simulink library "outp"  (R2021b)
(part 8 of 10)

  VTPM_LRSensorMode_flg_Inproc : FVT_lib/outp/OverrideAndLimit  SystemSampleTime=-1  VariantActivationTime=update diagram  Latency=0  AutoFrameSizeCalculation=off
      link override Signal_Limit/_maxval: Value=KOUTP_LRSensorMode_flg_maxval
      link override Signal_Limit/_minval: Value=KOUTP_LRSensorMode_flg_minval
      link override Signal_Override/_ovrdflg: Value=KOUTP_LRSensorMode_flg_ovrdflg
      link override Signal_Override/_ovrdval: Value=KOUTP_LRSensorMode_flg_ovrdval
  VTPM_LRWheelDebug_flg_Inproc : FVT_lib/outp/OverrideAndLimit  SystemSampleTime=-1  VariantActivationTime=update diagram  Latency=0  AutoFrameSizeCalculation=off
      link override Signal_Limit/_maxval: Value=KOUTP_LRWheelDebug_flg_maxval
      link override Signal_Limit/_minval: Value=KOUTP_LRWheelDebug_flg_minval
      link override Signal_Override/_ovrdflg: Value=KOUTP_LRWheelDebug_flg_ovrdflg
      link override Signal_Override/_ovrdval: Value=KOUTP_LRWheelDebug_flg_ovrdval
  VTPM_LRWheelPSW_raw8_Inproc : FVT_lib/outp/OverrideAndLimit  SystemSampleTime=-1  VariantActivationTime=update diagram  Latency=0  AutoFrameSizeCalculation=off
      link override Signal_Limit/_maxval: Value=KOUTP_LRWheelPSW_raw8_maxval
      link override Signal_Limit/_minval: Value=KOUTP_LRWheelPSW_raw8_minval
      link override Signal_Override/_ovrdflg: Value=KOUTP_LRWheelPSW_raw8_ovrdflg
      link override Signal_Override/_ovrdval: Value=KOUTP_LRWheelPSW_raw8_ovrdval
  VTPM_LRWheelPress_raw8_Inproc : FVT_lib/outp/OverrideAndLimit  SystemSampleTime=-1  VariantActivationTime=update diagram  Latency=0  AutoFrameSizeCalculation=off
      link override Signal_Limit/_maxval: Value=KOUTP_LRWheelPress_raw8_maxval
      link override Signal_Limit/_minval: Value=KOUTP_LRWheelPress_raw8_minval
      link override Signal_Override/_ovrdflg: Value=KOUTP_LRWheelPress_raw8_ovrdflg
      link override Signal_Override/_ovrdval: Value=KOUTP_LRWheelPress_raw8_ovrdval
  VTPM_LRWheelTemp_C_Inproc : FVT_lib/outp/OverrideAndLimit  SystemSampleTime=-1  VariantActivationTime=update diagram  Latency=0  AutoFrameSizeCalculation=off
      link override Signal_Limit/_maxval: Value=KOUTP_LRWheelTemp_C_maxval
      link override Signal_Limit/_minval: Value=KOUTP_LRWheelTemp_C_minval
      link override Signal_Override/_ovrdflg: Value=KOUTP_LRWheelTemp_C_ovrdflg
      link override Signal_Override/_ovrdval: Value=KOUTP_LRWheelTemp_C_ovrdval
  VTPM_LRWheelTmpIndi_flg_Inproc : FVT_lib/outp/OverrideAndLimit  SystemSampleTime=-1  VariantActivationTime=update diagram  Latency=0  AutoFrameSizeCalculation=off
      link override Signal_Limit/_maxval: Value=KOUTP_LRWheelTmpIndi_flg_maxval
      link override Signal_Limit/_minval: Value=KOUTP_LRWheelTmpIndi_flg_minval
      link override Signal_Override/_ovrdflg: Value=KOUTP_LRWheelTmpIndi_flg_ovrdflg
      link override Signal_Override/_ovrdval: Value=KOUTP_LRWheelTmpIndi_flg_ovrdval
  VTPM_ModelVersionChksum_raw_Inproc : FVT_lib/outp/OverrideAndLimit  SystemSampleTime=-1  VariantActivationTime=update diagram  Latency=0  AutoFrameSizeCalculation=off
      link override Signal_Limit/_maxval: Value=KOUTP_ModelVersionChksum_raw_maxval
      link override Signal_Limit/_minval: Value=KOUTP_ModelVersionChksum_raw_minval
      link override Signal_Override/_ovrdflg: Value=KOUTP_ModelVersionChksum_raw_ovrdflg
      link override Signal_Override/_ovrdval: Value=KOUTP_ModelVersionChksum_raw_ovrdval
  VTPM_ModelVersion_raw_Inproc : FVT_lib/outp/OverrideAndLimit  SystemSampleTime=-1  VariantActivationTime=update diagram  Latency=0  AutoFrameSizeCalculation=off
      link override Signal_Limit/_maxval: Value=KOUTP_ModelVersion_raw_maxval
      link override Signal_Limit/_minval: Value=KOUTP_ModelVersion_raw_minval
      link override Signal_Override/_ovrdflg: Value=KOUTP_ModelVersion_raw_ovrdflg
      link override Signal_Override/_ovrdval: Value=KOUTP_ModelVersion_raw_ovrdval
  VTPM_Prepresstempvalid_enum_Inproc : FVT_lib/outp/OverrideAndLimit  SystemSampleTime=-1  VariantActivationTime=update diagram  Latency=0  AutoFrameSizeCalculation=off
      link override Signal_Limit/_maxval: Value=KOUTP_Prepresstempvalid_enum_maxval
      link override Signal_Limit/_minval: Value=KOUTP_Prepresstempvalid_enum_minval
      link override Signal_Override/_ovrdflg: Value=KOUTP_Prepresstempvalid_enum_ovrdflg
      link override Signal_Override/_ovrdval: Value=KOUTP_Prepresstempvalid_enum_ovrdval
  VTPM_RFBatWarn_flg_Inproc : FVT_lib/outp/OverrideAndLimit  SystemSampleTime=-1  VariantActivationTime=update diagram  Latency=0  AutoFrameSizeCalculation=off
      link override Signal_Limit/_maxval: Value=KOUTP_RFBatWarn_flg_maxval
      link override Signal_Limit/_minval: Value=KOUTP_RFBatWarn_flg_minval
      link override Signal_Override/_ovrdflg: Value=KOUTP_RFBatWarn_flg_ovrdflg
      link override Signal_Override/_ovrdval: Value=KOUTP_RFBatWarn_flg_ovrdval
  VTPM_RFP20_raw8_Inproc : FVT_lib/outp/OverrideAndLimit  SystemSampleTime=-1  VariantActivationTime=update diagram  Latency=0  AutoFrameSizeCalculation=off
      link override Signal_Limit/_maxval: Value=KOUTP_RFP20_raw8_maxval
      link override Signal_Limit/_minval: Value=KOUTP_RFP20_raw8_minval
      link override Signal_Override/_ovrdflg: Value=KOUTP_RFP20_raw8_ovrdflg
      link override Signal_Override/_ovrdval: Value=KOUTP_RFP20_raw8_ovrdval
  VTPM_RFPind_enum_Inproc : FVT_lib/outp/OverrideAndLimit  SystemSampleTime=-1  VariantActivationTime=update diagram  Latency=0  AutoFrameSizeCalculation=off
      link override Signal_Limit/_maxval: Value=KOUTP_RFPind_enum_maxval
      link override Signal_Limit/_minval: Value=KOUTP_RFPind_enum_minval
      link override Signal_Override/_ovrdflg: Value=KOUTP_RFPind_enum_ovrdflg
      link override Signal_Override/_ovrdval: Value=KOUTP_RFPind_enum_ovrdval
  VTPM_RFPressIndi_enum_Inproc : FVT_lib/outp/OverrideAndLimit  SystemSampleTime=-1  VariantActivationTime=update diagram  Latency=0  AutoFrameSizeCalculation=off
      link override Signal_Limit/_maxval: Value=KOUTP_RFPressIndi_enum_maxval
      link override Signal_Limit/_minval: Value=KOUTP_RFPressIndi_enum_minval
      link override Signal_Override/_ovrdflg: Value=KOUTP_RFPressIndi_enum_ovrdflg
      link override Signal_Override/_ovrdval: Value=KOUTP_RFPressIndi_enum_ovrdval
  VTPM_RFSensorFail_flg_Inproc : FVT_lib/outp/OverrideAndLimit  SystemSampleTime=-1  VariantActivationTime=update diagram  Latency=0  AutoFrameSizeCalculation=off
      link override Signal_Limit/_maxval: Value=KOUTP_RFSensorFail_flg_maxval
      link override Signal_Limit/_minval: Value=KOUTP_RFSensorFail_flg_minval
      link override Signal_Override/_ovrdflg: Value=KOUTP_RFSensorFail_flg_ovrdflg
      link override Signal_Override/_ovrdval: Value=KOUTP_RFSensorFail_flg_ovrdval
  VTPM_RFSensorMode_flg_Inproc : FVT_lib/outp/OverrideAndLimit  SystemSampleTime=-1  VariantActivationTime=update diagram  Latency=0  AutoFrameSizeCalculation=off
      link override Signal_Limit/_maxval: Value=KOUTP_RFSensorMode_flg_maxval
      link override Signal_Limit/_minval: Value=KOUTP_RFSensorMode_flg_minval
      link override Signal_Override/_ovrdflg: Value=KOUTP_RFSensorMode_flg_ovrdflg
      link override Signal_Override/_ovrdval: Value=KOUTP_RFSensorMode_flg_ovrdval
  VTPM_RFWheelDebug_flg_Inproc : FVT_lib/outp/OverrideAndLimit  SystemSampleTime=-1  VariantActivationTime=update diagram  Latency=0  AutoFrameSizeCalculation=off
      link override Signal_Limit/_maxval: Value=KOUTP_RFWheelDebug_flg_maxval
      link override Signal_Limit/_minval: Value=KOUTP_RFWheelDebug_flg_minval
      link override Signal_Override/_ovrdflg: Value=KOUTP_RFWheelDebug_flg_ovrdflg
      link override Signal_Override/_ovrdval: Value=KOUTP_RFWheelDebug_flg_ovrdval
  VTPM_RFWheelPSW_raw8_Inproc : FVT_lib/outp/OverrideAndLimit  SystemSampleTime=-1  VariantActivationTime=update diagram  Latency=0  AutoFrameSizeCalculation=off
      link override Signal_Limit/_maxval: Value=KOUTP_RFWheelPSW_raw8_maxval
      link override Signal_Limit/_minval: Value=KOUTP_RFWheelPSW_raw8_minval
      link override Signal_Override/_ovrdflg: Value=KOUTP_RFWheelPSW_raw8_ovrdflg
      link override Signal_Override/_ovrdval: Value=KOUTP_RFWheelPSW_raw8_ovrdval
  VTPM_RFWheelPress_raw8_Inproc : FVT_lib/outp/OverrideAndLimit  SystemSampleTime=-1  VariantActivationTime=update diagram  Latency=0  AutoFrameSizeCalculation=off
      link override Signal_Limit/_maxval: Value=KOUTP_RFWheelPress_raw8_maxval
      link override Signal_Limit/_minval: Value=KOUTP_RFWheelPress_raw8_minval
      link override Signal_Override/_ovrdflg: Value=KOUTP_RFWheelPress_raw8_ovrdflg
      link override Signal_Override/_ovrdval: Value=KOUTP_RFWheelPress_raw8_ovrdval
  VTPM_RFWheelTemp_C_Inproc : FVT_lib/outp/OverrideAndLimit  SystemSampleTime=-1  VariantActivationTime=update diagram  Latency=0  AutoFrameSizeCalculation=off
      link override Signal_Limit/_maxval: Value=KOUTP_RFWheelTemp_C_maxval
      link override Signal_Limit/_minval: Value=KOUTP_RFWheelTemp_C_minval
      link override Signal_Override/_ovrdflg: Value=KOUTP_RFWheelTemp_C_ovrdflg
      link override Signal_Override/_ovrdval: Value=KOUTP_RFWheelTemp_C_ovrdval
  VTPM_RFWheelTmpIndi_flg_Inproc : FVT_lib/outp/OverrideAndLimit  SystemSampleTime=-1  VariantActivationTime=update diagram  Latency=0  AutoFrameSizeCalculation=off
      link override Signal_Limit/_maxval: Value=KOUTP_RFWheelTmpIndi_flg_maxval
      link override Signal_Limit/_minval: Value=KOUTP_RFWheelTmpIndi_flg_minval
      link override Signal_Override/_ovrdflg: Value=KOUTP_RFWheelTmpIndi_flg_ovrdflg
      link override Signal_Override/_ovrdval: Value=KOUTP_RFWheelTmpIndi_flg_ovrdval
  VTPM_RRBatWarn_flg_Inproc : FVT_lib/outp/OverrideAndLimit  SystemSampleTime=-1  VariantActivationTime=update diagram  Latency=0  AutoFrameSizeCalculation=off
      link override Signal_Limit/_maxval: Value=KOUTP_RRBatWarn_flg_maxval
      link override Signal_Limit/_minval: Value=KOUTP_RRBatWarn_flg_minval
      link override Signal_Override/_ovrdflg: Value=KOUTP_RRBatWarn_flg_ovrdflg
      link override Signal_Override/_ovrdval: Value=KOUTP_RRBatWarn_flg_ovrdval
  VTPM_RRP20_raw8_Inproc : FVT_lib/outp/OverrideAndLimit  SystemSampleTime=-1  VariantActivationTime=update diagram  Latency=0  AutoFrameSizeCalculation=off
      link override Signal_Limit/_maxval: Value=KOUTP_RRP20_raw8_maxval
      link override Signal_Limit/_minval: Value=KOUTP_RRP20_raw8_minval
      link override Signal_Override/_ovrdflg: Value=KOUTP_RRP20_raw8_ovrdflg
      link override Signal_Override/_ovrdval: Value=KOUTP_RRP20_raw8_ovrdval
  VTPM_RRPindi_enum_Inproc : FVT_lib/outp/OverrideAndLimit  SystemSampleTime=-1  VariantActivationTime=update diagram  Latency=0  AutoFrameSizeCalculation=off
      link override Signal_Limit/_maxval: Value=KOUTP_RRPindi_enum_maxval
      link override Signal_Limit/_minval: Value=KOUTP_RRPindi_enum_minval
      link override Signal_Override/_ovrdflg: Value=KOUTP_RRPindi_enum_ovrdflg
      link override Signal_Override/_ovrdval: Value=KOUTP_RRPindi_enum_ovrdval
  VTPM_RRPressIndi_enum_Inproc : FVT_lib/outp/OverrideAndLimit  SystemSampleTime=-1  VariantActivationTime=update diagram  Latency=0  AutoFrameSizeCalculation=off
      link override Signal_Limit/_maxval: Value=KOUTP_RRPressIndi_enum_maxval
      link override Signal_Limit/_minval: Value=KOUTP_RRPressIndi_enum_minval
      link override Signal_Override/_ovrdflg: Value=KOUTP_RRPressIndi_enum_ovrdflg
      link override Signal_Override/_ovrdval: Value=KOUTP_RRPressIndi_enum_ovrdval
  VTPM_RRSensorFail_flg_Inproc : FVT_lib/outp/OverrideAndLimit  SystemSampleTime=-1  VariantActivationTime=update diagram  Latency=0  AutoFrameSizeCalculation=off
      link override Signal_Limit/_maxval: Value=KOUTP_RRSensorFail_flg_maxval
      link override Signal_Limit/_minval: Value=KOUTP_RRSensorFail_flg_minval
      link override Signal_Override/_ovrdflg: Value=KOUTP_RRSensorFail_flg_ovrdflg
      link override Signal_Override/_ovrdval: Value=KOUTP_RRSensorFail_flg_ovrdval
  VTPM_RRSensorMode_flg_Inproc : FVT_lib/outp/OverrideAndLimit  SystemSampleTime=-1  VariantActivationTime=update diagram  Latency=0  AutoFrameSizeCalculation=off
      link override Signal_Limit/_maxval: Value=KOUTP_RRSensorMode_flg_maxval
      link override Signal_Limit/_minval: Value=KOUTP_RRSensorMode_flg_minval
      link override Signal_Override/_ovrdflg: Value=KOUTP_RRSensorMode_flg_ovrdflg
      link override Signal_Override/_ovrdval: Value=KOUTP_RRSensorMode_flg_ovrdval
  VTPM_RRWheelDebug_flg_Inproc : FVT_lib/outp/OverrideAndLimit  SystemSampleTime=-1  VariantActivationTime=update diagram  Latency=0  AutoFrameSizeCalculation=off
      link override Signal_Limit/_maxval: Value=KOUTP_RRWheelDebug_flg_maxval
      link override Signal_Limit/_minval: Value=KOUTP_RRWheelDebug_flg_minval
      link override Signal_Override/_ovrdflg: Value=KOUTP_RRWheelDebug_flg_ovrdflg
      link override Signal_Override/_ovrdval: Value=KOUTP_RRWheelDebug_flg_ovrdval
  VTPM_RRWheelPSW_raw8_Inproc : FVT_lib/outp/OverrideAndLimit  SystemSampleTime=-1  VariantActivationTime=update diagram  Latency=0  AutoFrameSizeCalculation=off
      link override Signal_Limit/_maxval: Value=KOUTP_RRWheelPSW_raw8_maxval
      link override Signal_Limit/_minval: Value=KOUTP_RRWheelPSW_raw8_minval
      link override Signal_Override/_ovrdflg: Value=KOUTP_RRWheelPSW_raw8_ovrdflg
      link override Signal_Override/_ovrdval: Value=KOUTP_RRWheelPSW_raw8_ovrdval
  VTPM_RRWheelPress_raw8_Inproc : FVT_lib/outp/OverrideAndLimit  SystemSampleTime=-1  VariantActivationTime=update diagram  Latency=0  AutoFrameSizeCalculation=off
      link override Signal_Limit/_maxval: Value=KOUTP_RRWheelPress_raw8_maxval
      link override Signal_Limit/_minval: Value=KOUTP_RRWheelPress_raw8_minval
      link override Signal_Override/_ovrdflg: Value=KOUTP_RRWheelPress_raw8_ovrdflg
      link override Signal_Override/_ovrdval: Value=KOUTP_RRWheelPress_raw8_ovrdval
  VTPM_RRWheelTemp_C_Inproc : FVT_lib/outp/OverrideAndLimit  SystemSampleTime=-1  VariantActivationTime=update diagram  Latency=0  AutoFrameSizeCalculation=off
      link override Signal_Limit/_maxval: Value=KOUTP_RRWheelTemp_C_maxval
      link override Signal_Limit/_minval: Value=KOUTP_RRWheelTemp_C_minval
      link override Signal_Override/_ovrdflg: Value=KOUTP_RRWheelTemp_C_ovrdflg
      link override Signal_Override/_ovrdval: Value=KOUTP_RRWheelTemp_C_ovrdval
  VTPM_RRWheelTmpIndi_flg_Inproc : FVT_lib/outp/OverrideAndLimit  SystemSampleTime=-1  VariantActivationTime=update diagram  Latency=0  AutoFrameSizeCalculation=off
      link override Signal_Limit/_maxval: Value=KOUTP_RRWheelTmpIndi_flg_maxval
      link override Signal_Limit/_minval: Value=KOUTP_RRWheelTmpIndi_flg_minval
      link override Signal_Override/_ovrdflg: Value=KOUTP_RRWheelTmpIndi_flg_ovrdflg
      link override Signal_Override/_ovrdval: Value=KOUTP_RRWheelTmpIndi_flg_ovrdval
  VTPM_S1ID_raw32_Inproc : FVT_lib/outp/OverrideAndLimit  SystemSampleTime=-1  VariantActivationTime=update diagram  Latency=0  AutoFrameSizeCalculation=off
      link override Signal_Limit/_maxval: Value=KOUTP_S1ID_raw32_maxval
      link override Signal_Limit/_minval: Value=KOUTP_S1ID_raw32_minval
      link override Signal_Override/_ovrdflg: Value=KOUTP_S1ID_raw32_ovrdflg
      link override Signal_Override/_ovrdval: Value=KOUTP_S1ID_raw32_ovrdval
  VTPM_S1L_enum_Inproc : FVT_lib/outp/OverrideAndLimit  SystemSampleTime=-1  VariantActivationTime=update diagram  Latency=0  AutoFrameSizeCalculation=off
      link override Signal_Limit/_maxval: Value=KOUTP_S1L_enum_maxval
      link override Signal_Limit/_minval: Value=KOUTP_S1L_enum_minval
      link override Signal_Override/_ovrdflg: Value=KOUTP_S1L_enum_ovrdflg
      link override Signal_Override/_ovrdval: Value=KOUTP_S1L_enum_ovrdval
  VTPM_S1WheelDebugALTU_pct_Inproc : FVT_lib/outp/OverrideAndLimit  SystemSampleTime=-1  VariantActivationTime=update diagram  Latency=0  AutoFrameSizeCalculation=off
      link override Signal_Limit/_maxval: Value=KOUTP_S1WheelDebugALTU_pct_maxval
      link override Signal_Limit/_minval: Value=KOUTP_S1WheelDebugALTU_pct_minval
      link override Signal_Override/_ovrdflg: Value=KOUTP_S1WheelDebugALTU_pct_ovrdflg
      link override Signal_Override/_ovrdval: Value=KOUTP_S1WheelDebugALTU_pct_ovrdval
  VTPM_S2ID_raw32_Inproc : FVT_lib/outp/OverrideAndLimit  SystemSampleTime=-1  VariantActivationTime=update diagram  Latency=0  AutoFrameSizeCalculation=off
      link override Signal_Limit/_maxval: Value=KOUTP_S2ID_raw32_maxval
      link override Signal_Limit/_minval: Value=KOUTP_S2ID_raw32_minval
      link override Signal_Override/_ovrdflg: Value=KOUTP_S2ID_raw32_ovrdflg
      link override Signal_Override/_ovrdval: Value=KOUTP_S2ID_raw32_ovrdval
  VTPM_S2L_enum_Inproc : FVT_lib/outp/OverrideAndLimit  SystemSampleTime=-1  VariantActivationTime=update diagram  Latency=0  AutoFrameSizeCalculation=off
      link override Signal_Limit/_maxval: Value=KOUTP_S2L_enum_maxval
      link override Signal_Limit/_minval: Value=KOUTP_S2L_enum_minval
      link override Signal_Override/_ovrdflg: Value=KOUTP_S2L_enum_ovrdflg
      link override Signal_Override/_ovrdval: Value=KOUTP_S2L_enum_ovrdval
  VTPM_S2WheelDebugALTU_pct_Inproc : FVT_lib/outp/OverrideAndLimit  SystemSampleTime=-1  VariantActivationTime=update diagram  Latency=0  AutoFrameSizeCalculation=off
      link override Signal_Limit/_maxval: Value=KOUTP_S2WheelDebugALTU_pct_maxval
      link override Signal_Limit/_minval: Value=KOUTP_S2WheelDebugALTU_pct_minval
      link override Signal_Override/_ovrdflg: Value=KOUTP_S2WheelDebugALTU_pct_ovrdflg
      link override Signal_Override/_ovrdval: Value=KOUTP_S2WheelDebugALTU_pct_ovrdval
  VTPM_S3ID_raw32_Inproc : FVT_lib/outp/OverrideAndLimit  SystemSampleTime=-1  VariantActivationTime=update diagram  Latency=0  AutoFrameSizeCalculation=off
      link override Signal_Limit/_maxval: Value=KOUTP_S3ID_raw32_maxval
      link override Signal_Limit/_minval: Value=KOUTP_S3ID_raw32_minval
      link override Signal_Override/_ovrdflg: Value=KOUTP_S3ID_raw32_ovrdflg
      link override Signal_Override/_ovrdval: Value=KOUTP_S3ID_raw32_ovrdval
  VTPM_S3L_enum_Inproc : FVT_lib/outp/OverrideAndLimit  SystemSampleTime=-1  VariantActivationTime=update diagram  Latency=0  AutoFrameSizeCalculation=off
      link override Signal_Limit/_maxval: Value=KOUTP_S3L_enum_maxval
      link override Signal_Limit/_minval: Value=KOUTP_S3L_enum_minval
      link override Signal_Override/_ovrdflg: Value=KOUTP_S3L_enum_ovrdflg
      link override Signal_Override/_ovrdval: Value=KOUTP_S3L_enum_ovrdval
  VTPM_S3WheelDebugALTU_pct_Inproc : FVT_lib/outp/OverrideAndLimit  SystemSampleTime=-1  VariantActivationTime=update diagram  Latency=0  AutoFrameSizeCalculation=off
      link override Signal_Limit/_maxval: Value=KOUTP_S3WheelDebugALTU_pct_maxval
      link override Signal_Limit/_minval: Value=KOUTP_S3WheelDebugALTU_pct_minval
      link override Signal_Override/_ovrdflg: Value=KOUTP_S3WheelDebugALTU_pct_ovrdflg
      link override Signal_Override/_ovrdval: Value=KOUTP_S3WheelDebugALTU_pct_ovrdval
  VTPM_S4ID_raw32_Inproc : FVT_lib/outp/OverrideAndLimit  SystemSampleTime=-1  VariantActivationTime=update diagram  Latency=0  AutoFrameSizeCalculation=off
      link override Signal_Limit/_maxval: Value=KOUTP_S4ID_raw32_maxval
      link override Signal_Limit/_minval: Value=KOUTP_S4ID_raw32_minval
      link override Signal_Override/_ovrdflg: Value=KOUTP_S4ID_raw32_ovrdflg
      link override Signal_Override/_ovrdval: Value=KOUTP_S4ID_raw32_ovrdval
  VTPM_S4L_enum_Inproc : FVT_lib/outp/OverrideAndLimit  SystemSampleTime=-1  VariantActivationTime=update diagram  Latency=0  AutoFrameSizeCalculation=off
      link override Signal_Limit/_maxval: Value=KOUTP_S4L_enum_maxval
      link override Signal_Limit/_minval: Value=KOUTP_S4L_enum_minval
      link override Signal_Override/_ovrdflg: Value=KOUTP_S4L_enum_ovrdflg
      link override Signal_Override/_ovrdval: Value=KOUTP_S4L_enum_ovrdval
  VTPM_S4WheelDebugALTU_pct_Inproc : FVT_lib/outp/OverrideAndLimit  SystemSampleTime=-1  VariantActivationTime=update diagram  Latency=0  AutoFrameSizeCalculation=off
      link override Signal_Limit/_maxval: Value=KOUTP_S4WheelDebugALTU_pct_maxval
      link override Signal_Limit/_minval: Value=KOUTP_S4WheelDebugALTU_pct_minval
      link override Signal_Override/_ovrdflg: Value=KOUTP_S4WheelDebugALTU_pct_ovrdflg
      link override Signal_Override/_ovrdval: Value=KOUTP_S4WheelDebugALTU_pct_ovrdval
  VTPM_SetIDLoc_flg_Inproc : FVT_lib/outp/OverrideAndLimit  SystemSampleTime=-1  VariantActivationTime=update diagram  Latency=0  AutoFrameSizeCalculation=off
      link override Signal_Limit/_maxval: Value=KOUTP_SetIDLoc_flg_maxval
      link override Signal_Limit/_minval: Value=KOUTP_SetIDLoc_flg_minval
      link override Signal_Override/_ovrdflg: Value=KOUTP_SetIDLoc_flg_ovrdflg
      link override Signal_Override/_ovrdval: Value=KOUTP_SetIDLoc_flg_ovrdval
  VTPM_TPMSCaliButtAllow_flg_Inproc : FVT_lib/outp/OverrideAndLimit  SystemSampleTime=-1  VariantActivationTime=update diagram  Latency=0  AutoFrameSizeCalculation=off
      link override Signal_Limit/_maxval: Value=KOUTP_TPMSCaliButtAllow_flg_maxval
      link override Signal_Limit/_minval: Value=KOUTP_TPMSCaliButtAllow_flg_minval
      link override Signal_Override/_ovrdflg: Value=KOUTP_TPMSCaliButtAllow_flg_ovrdflg
      link override Signal_Override/_ovrdval: Value=KOUTP_TPMSCaliButtAllow_flg_ovrdval
  VTPM_TPMSResButtAllow_flg_Inproc : FVT_lib/outp/OverrideAndLimit  SystemSampleTime=-1  VariantActivationTime=update diagram  Latency=0  AutoFrameSizeCalculation=off
      link override Signal_Limit/_maxval: Value=KOUTP_TPMSResButtAllow_flg_maxval
      link override Signal_Limit/_minval: Value=KOUTP_TPMSResButtAllow_flg_minval
      link override Signal_Override/_ovrdflg: Value=KOUTP_TPMSResButtAllow_flg_ovrdflg
      link override Signal_Override/_ovrdval: Value=KOUTP_TPMSResButtAllow_flg_ovrdval
  VTPM_TPMSResButt_flg_Inproc : FVT_lib/outp/OverrideAndLimit  SystemSampleTime=-1  VariantActivationTime=update diagram  Latency=0  AutoFrameSizeCalculation=off
      link override Signal_Limit/_maxval: Value=KOUTP_TPMSResButt_flg_maxval
      link override Signal_Limit/_minval: Value=KOUTP_TPMSResButt_flg_minval
      link override Signal_Override/_ovrdflg: Value=KOUTP_TPMSResButt_flg_ovrdflg
      link override Signal_Override/_ovrdval: Value=KOUTP_TPMSResButt_flg_ovrdval
  VTPM_TPMSSensorIDRegStart_flg_Inproc : FVT_lib/outp/OverrideAndLimit  SystemSampleTime=-1  VariantActivationTime=update diagram  Latency=0  AutoFrameSizeCalculation=off
      link override Signal_Limit/_maxval: Value=KOUTP_TPMSSensorIDRegStart_flg_maxval
      link override Signal_Limit/_minval: Value=KOUTP_TPMSSensorIDRegStart_flg_minval
      link override Signal_Override/_ovrdflg: Value=KOUTP_TPMSSensorIDRegStart_flg_ovrdflg
      link override Signal_Override/_ovrdval: Value=KOUTP_TPMSSensorIDRegStart_flg_ovrdval
  VTPM_TPMSStorge_flg_Inproc : FVT_lib/outp/OverrideAndLimit  SystemSampleTime=-1  VariantActivationTime=update diagram  Latency=0  AutoFrameSizeCalculation=off
      link override Signal_Limit/_maxval: Value=KOUTP_TPMSStorge_flg_maxval
      link override Signal_Limit/_minval: Value=KOUTP_TPMSStorge_flg_minval
      link override Signal_Override/_ovrdflg: Value=KOUTP_TPMSStorge_flg_ovrdflg
      link override Signal_Override/_ovrdval: Value=KOUTP_TPMSStorge_flg_ovrdval
  VTPM_TPMSTLCmd_flg_Inproc : FVT_lib/outp/OverrideAndLimit  SystemSampleTime=-1  VariantActivationTime=update diagram  Latency=0  AutoFrameSizeCalculation=off
      link override Signal_Limit/_maxval: Value=KOUTP_TPMSTLCmd_flg_maxval
      link override Signal_Limit/_minval: Value=KOUTP_TPMSTLCmd_flg_minval
      link override Signal_Override/_ovrdflg: Value=KOUTP_TPMSTLCmd_flg_ovrdflg
      link override Signal_Override/_ovrdval: Value=KOUTP_TPMSTLCmd_flg_ovrdval
  VTPM_TPMSWarnIndi_enum_Inproc : FVT_lib/outp/OverrideAndLimit  SystemSampleTime=-1  VariantActivationTime=update diagram  Latency=0  AutoFrameSizeCalculation=off
      link override Signal_Limit/_maxval: Value=KOUTP_TPMSWarnIndi_enum_maxval
      link override Signal_Limit/_minval: Value=KOUTP_TPMSWarnIndi_enum_minval
      link override Signal_Override/_ovrdflg: Value=KOUTP_TPMSWarnIndi_enum_ovrdflg
      link override Signal_Override/_ovrdval: Value=KOUTP_TPMSWarnIndi_enum_ovrdval
  VTPM_WriteChkLFID_raw_Inproc : FVT_lib/outp/OverrideAndLimit  SystemSampleTime=-1  VariantActivationTime=update diagram  Latency=0  AutoFrameSizeCalculation=off
      link override Signal_Limit/_maxval: Value=KOUTP_WriteChkLFID_raw_maxval
      link override Signal_Limit/_minval: Value=KOUTP_WriteChkLFID_raw_minval
      link override Signal_Override/_ovrdflg: Value=KOUTP_WriteChkLFID_raw_ovrdflg
      link override Signal_Override/_ovrdval: Value=KOUTP_WriteChkLFID_raw_ovrdval
  VTPM_WriteChkLRID_raw_Inproc : FVT_lib/outp/OverrideAndLimit  SystemSampleTime=-1  VariantActivationTime=update diagram  Latency=0  AutoFrameSizeCalculation=off
      link override Signal_Limit/_maxval: Value=KOUTP_WriteChkLRID_raw_maxval
      link override Signal_Limit/_minval: Value=KOUTP_WriteChkLRID_raw_minval
      link override Signal_Override/_ovrdflg: Value=KOUTP_WriteChkLRID_raw_ovrdflg
      link override Signal_Override/_ovrdval: Value=KOUTP_WriteChkLRID_raw_ovrdval
  VTPM_WriteChkRFID_raw_Inproc : FVT_lib/outp/OverrideAndLimit  SystemSampleTime=-1  VariantActivationTime=update diagram  Latency=0  AutoFrameSizeCalculation=off
      link override Signal_Limit/_maxval: Value=KOUTP_WriteChkRFID_raw_maxval
      link override Signal_Limit/_minval: Value=KOUTP_WriteChkRFID_raw_minval
      link override Signal_Override/_ovrdflg: Value=KOUTP_WriteChkRFID_raw_ovrdflg
      link override Signal_Override/_ovrdval: Value=KOUTP_WriteChkRFID_raw_ovrdval
  VTPM_WriteChkRRID_raw_Inproc : FVT_lib/outp/OverrideAndLimit  SystemSampleTime=-1  VariantActivationTime=update diagram  Latency=0  AutoFrameSizeCalculation=off
      link override Signal_Limit/_maxval: Value=KOUTP_WriteChkRRID_raw_maxval
      link override Signal_Limit/_minval: Value=KOUTP_WriteChkRRID_raw_minval
      link override Signal_Override/_ovrdflg: Value=KOUTP_WriteChkRRID_raw_ovrdflg
      link override Signal_Override/_ovrdval: Value=KOUTP_WriteChkRRID_raw_ovrdval
  VTPM_WriteChkfinLFID_raw_Inproc : FVT_lib/outp/OverrideAndLimit  SystemSampleTime=-1  VariantActivationTime=update diagram  Latency=0  AutoFrameSizeCalculation=off
      link override Signal_Limit/_maxval: Value=KOUTP_WriteChkfinLFID_raw_maxval
      link override Signal_Limit/_minval: Value=KOUTP_WriteChkfinLFID_raw_minval
      link override Signal_Override/_ovrdflg: Value=KOUTP_WriteChkfinLFID_raw_ovrdflg
      link override Signal_Override/_ovrdval: Value=KOUTP_WriteChkfinLFID_raw_ovrdval
  VTPM_WriteChkfinLRID_raw_Inproc : FVT_lib/outp/OverrideAndLimit  SystemSampleTime=-1  VariantActivationTime=update diagram  Latency=0  AutoFrameSizeCalculation=off
      link override Signal_Limit/_maxval: Value=KOUTP_WriteChkfinLRID_raw_maxval
      link override Signal_Limit/_minval: Value=KOUTP_WriteChkfinLRID_raw_minval
      link override Signal_Override/_ovrdflg: Value=KOUTP_WriteChkfinLRID_raw_ovrdflg
      link override Signal_Override/_ovrdval: Value=KOUTP_WriteChkfinLRID_raw_ovrdval
  VTPM_WriteChkfinRFID_raw_Inproc : FVT_lib/outp/OverrideAndLimit  SystemSampleTime=-1  VariantActivationTime=update diagram  Latency=0  AutoFrameSizeCalculation=off
      link override Signal_Limit/_maxval: Value=KOUTP_WriteChkfinRFID_raw_maxval
      link override Signal_Limit/_minval: Value=KOUTP_WriteChkfinRFID_raw_minval
      link override Signal_Override/_ovrdflg: Value=KOUTP_WriteChkfinRFID_raw_ovrdflg
      link override Signal_Override/_ovrdval: Value=KOUTP_WriteChkfinRFID_raw_ovrdval
  VTPM_WriteChkfinRRID_raw_Inproc : FVT_lib/outp/OverrideAndLimit  SystemSampleTime=-1  VariantActivationTime=update diagram  Latency=0  AutoFrameSizeCalculation=off
      link override Signal_Limit/_maxval: Value=KOUTP_WriteChkfinRRID_raw_maxval
      link override Signal_Limit/_minval: Value=KOUTP_WriteChkfinRRID_raw_minval
      link override Signal_Override/_ovrdflg: Value=KOUTP_WriteChkfinRRID_raw_ovrdflg
      link override Signal_Override/_ovrdval: Value=KOUTP_WriteChkfinRRID_raw_ovrdval
  VTPM_WritingCnt_enum_Inproc : FVT_lib/outp/OverrideAndLimit  SystemSampleTime=-1  VariantActivationTime=update diagram  Latency=0  AutoFrameSizeCalculation=off
      link override Signal_Limit/_maxval: Value=KOUTP_WritingCnt_enum_maxval
      link override Signal_Limit/_minval: Value=KOUTP_WritingCnt_enum_minval
      link override Signal_Override/_ovrdflg: Value=KOUTP_WritingCnt_enum_ovrdflg
      link override Signal_Override/_ovrdval: Value=KOUTP_WritingCnt_enum_ovrdval
  VTPM_unlearnSfailvalid_enum_Inproc : FVT_lib/outp/OverrideAndLimit  SystemSampleTime=-1  VariantActivationTime=update diagram  Latency=0  AutoFrameSizeCalculation=off
      link override Signal_Limit/_maxval: Value=KOUTP_unlearnSfailvalid_enum_maxval
      link override Signal_Limit/_minval: Value=KOUTP_unlearnSfailvalid_enum_minval
      link override Signal_Override/_ovrdflg: Value=KOUTP_unlearnSfailvalid_enum_ovrdflg
      link override Signal_Override/_ovrdval: Value=KOUTP_unlearnSfailvalid_enum_ovrdval
  VTPM_unlearnSfali_flg_Inproc : FVT_lib/outp/OverrideAndLimit  SystemSampleTime=-1  VariantActivationTime=update diagram  Latency=0  AutoFrameSizeCalculation=off
      link override Signal_Limit/_maxval: Value=KOUTP_unlearnSfali_flg_maxval
      link override Signal_Limit/_minval: Value=KOUTP_unlearnSfali_flg_minval
      link override Signal_Override/_ovrdflg: Value=KOUTP_unlearnSfali_flg_ovrdflg
      link override Signal_Override/_ovrdval: Value=KOUTP_unlearnSfali_flg_ovrdval
  VTQD_ActParkRequest_flg_Inproc : FVT_lib/outp/OverrideAndLimit  SystemSampleTime=-1  VariantActivationTime=update diagram  Latency=0  AutoFrameSizeCalculation=off
      link override Signal_Limit/_maxval: Value=KOUTP_ActParkRequest_flg_maxval
      link override Signal_Limit/_minval: Value=KOUTP_ActParkRequest_flg_minval
      link override Signal_Override/_ovrdflg: Value=KOUTP_ActParkRequest_flg_ovrdflg
      link override Signal_Override/_ovrdval: Value=KOUTP_ActParkRequest_flg_ovrdval
  VTQD_CreepON_flg_Inproc : FVT_lib/outp/OverrideAndLimit  SystemSampleTime=-1  VariantActivationTime=update diagram  Latency=0  AutoFrameSizeCalculation=off
      link override Signal_Limit/_maxval: Value=KOUTP_CreepON_flg_maxval
      link override Signal_Limit/_minval: Value=KOUTP_CreepON_flg_minval
      link override Signal_Override/_ovrdflg: Value=KOUTP_CreepON_flg_ovrdflg
      link override Signal_Override/_ovrdval: Value=KOUTP_CreepON_flg_ovrdval
  VTQD_DriveProtEn_flg_Inproc : FVT_lib/outp/OverrideAndLimit  SystemSampleTime=-1  VariantActivationTime=update diagram  Latency=0  AutoFrameSizeCalculation=off
      link override Signal_Limit/_maxval: Value=KOUTP_DriveProtEn_flg_maxval
      link override Signal_Limit/_minval: Value=KOUTP_DriveProtEn_flg_minval
      link override Signal_Override/_ovrdflg: Value=KOUTP_DriveProtEn_flg_ovrdflg
      link override Signal_Override/_ovrdval: Value=KOUTP_DriveProtEn_flg_ovrdval
  VTQD_DriverWhlTqDemFr_Nm_Inproc : FVT_lib/outp/OverrideAndLimit  SystemSampleTime=-1  VariantActivationTime=update diagram  Latency=0  AutoFrameSizeCalculation=off
      link override Signal_Limit/_maxval: Value=KOUTP_DriverWhlTqDemFr_Nm_maxval
      link override Signal_Limit/_minval: Value=KOUTP_DriverWhlTqDemFr_Nm_minval
      link override Signal_Override/_ovrdflg: Value=KOUTP_DriverWhlTqDemFr_Nm_ovrdflg
      link override Signal_Override/_ovrdval: Value=KOUTP_DriverWhlTqDemFr_Nm_ovrdval
  VTQD_DriverWhlTqDemRr_Nm_Inproc : FVT_lib/outp/OverrideAndLimit  SystemSampleTime=-1  VariantActivationTime=update diagram  Latency=0  AutoFrameSizeCalculation=off
      link override Signal_Limit/_maxval: Value=KOUTP_DriverWhlTqDemRr_Nm_maxval
      link override Signal_Limit/_minval: Value=KOUTP_DriverWhlTqDemRr_Nm_minval
      link override Signal_Override/_ovrdflg: Value=KOUTP_DriverWhlTqDemRr_Nm_ovrdflg
      link override Signal_Override/_ovrdval: Value=KOUTP_DriverWhlTqDemRr_Nm_ovrdval
  VTQD_EVDriveMode_enum_Inproc : FVT_lib/outp/OverrideAndLimit  SystemSampleTime=-1  VariantActivationTime=update diagram  Latency=0  AutoFrameSizeCalculation=off
      link override Signal_Limit/_maxval: Value=KOUTP_EVDriveMode_enum_maxval
      link override Signal_Limit/_minval: Value=KOUTP_EVDriveMode_enum_minval
      link override Signal_Override/_ovrdflg: Value=KOUTP_EVDriveMode_enum_ovrdflg
      link override Signal_Override/_ovrdval: Value=KOUTP_EVDriveMode_enum_ovrdval
  VTQD_EquivAccPedalSWSta_flg_Inproc : FVT_lib/outp/OverrideAndLimit  SystemSampleTime=-1  VariantActivationTime=update diagram  Latency=0  AutoFrameSizeCalculation=off
      link override Signal_Limit/_maxval: Value=KOUTP_EquivAccPedalSWSta_flg_maxval
      link override Signal_Limit/_minval: Value=KOUTP_EquivAccPedalSWSta_flg_minval
      link override Signal_Override/_ovrdflg: Value=KOUTP_EquivAccPedalSWSta_flg_ovrdflg
      link override Signal_Override/_ovrdval: Value=KOUTP_EquivAccPedalSWSta_flg_ovrdval
  VTQD_ExtDoorAllow_flg_Inproc : FVT_lib/outp/OverrideAndLimit  SystemSampleTime=-1  VariantActivationTime=update diagram  Latency=0  AutoFrameSizeCalculation=off
      link override Signal_Limit/_maxval: Value=KOUTP_ExtDoorAllow_flg_maxval
      link override Signal_Limit/_minval: Value=KOUTP_ExtDoorAllow_flg_minval
      link override Signal_Override/_ovrdflg: Value=KOUTP_ExtDoorAllow_flg_ovrdflg
      link override Signal_Override/_ovrdval: Value=KOUTP_ExtDoorAllow_flg_ovrdval
  VTQD_ExtShftAllow_flg_Inproc : FVT_lib/outp/OverrideAndLimit  SystemSampleTime=-1  VariantActivationTime=update diagram  Latency=0  AutoFrameSizeCalculation=off
      link override Signal_Limit/_maxval: Value=KOUTP_ExtShftAllow_flg_maxval
      link override Signal_Limit/_minval: Value=KOUTP_ExtShftAllow_flg_minval
      link override Signal_Override/_ovrdflg: Value=KOUTP_ExtShftAllow_flg_ovrdflg
      link override Signal_Override/_ovrdval: Value=KOUTP_ExtShftAllow_flg_ovrdval
  VTQD_ExternalTqAllow_flg_Inproc : FVT_lib/outp/OverrideAndLimit  SystemSampleTime=-1  VariantActivationTime=update diagram  Latency=0  AutoFrameSizeCalculation=off
      link override Signal_Limit/_maxval: Value=KOUTP_ExternalTqAllow_flg_maxval
      link override Signal_Limit/_minval: Value=KOUTP_ExternalTqAllow_flg_minval
      link override Signal_Override/_ovrdflg: Value=KOUTP_ExternalTqAllow_flg_ovrdflg
      link override Signal_Override/_ovrdval: Value=KOUTP_ExternalTqAllow_flg_ovrdval
  VTQD_FDCVCURegenMode_enum_Inproc : FVT_lib/outp/OverrideAndLimit  SystemSampleTime=-1  VariantActivationTime=update diagram  Latency=0  AutoFrameSizeCalculation=off
      link override Signal_Limit/_maxval: Value=KOUTP_FDCVCURegenMode_enum_maxval
      link override Signal_Limit/_minval: Value=KOUTP_FDCVCURegenMode_enum_minval
      link override Signal_Override/_ovrdflg: Value=KOUTP_FDCVCURegenMode_enum_ovrdflg
      link override Signal_Override/_ovrdval: Value=KOUTP_FDCVCURegenMode_enum_ovrdval
  VTQD_FrActvDmpDisabReq_flg_Inproc : FVT_lib/outp/OverrideAndLimit  SystemSampleTime=-1  VariantActivationTime=update diagram  Latency=0  AutoFrameSizeCalculation=off
      link override Signal_Limit/_maxval: Value=KOUTP_FrActvDmpDisabReq_flg_maxval
      link override Signal_Limit/_minval: Value=KOUTP_FrActvDmpDisabReq_flg_minval
      link override Signal_Override/_ovrdflg: Value=KOUTP_FrActvDmpDisabReq_flg_ovrdflg
      link override Signal_Override/_ovrdval: Value=KOUTP_FrActvDmpDisabReq_flg_ovrdval
  VTQD_FrEDUActTq_Nm_Inproc : FVT_lib/outp/OverrideAndLimit  SystemSampleTime=-1  VariantActivationTime=update diagram  Latency=0  AutoFrameSizeCalculation=off
      link override Signal_Limit/_maxval: Value=KOUTP_FrEDUActTq_Nm_maxval
      link override Signal_Limit/_minval: Value=KOUTP_FrEDUActTq_Nm_minval
      link override Signal_Override/_ovrdflg: Value=KOUTP_FrEDUActTq_Nm_ovrdflg
      link override Signal_Override/_ovrdval: Value=KOUTP_FrEDUActTq_Nm_ovrdval
  VTQD_FrEDUAvailBrkRgnTqV_flg_Inproc : FVT_lib/outp/OverrideAndLimit  SystemSampleTime=-1  VariantActivationTime=update diagram  Latency=0  AutoFrameSizeCalculation=off
      link override Signal_Limit/_maxval: Value=KOUTP_FrEDUAvailBrkRgnTqV_flg_maxval
      link override Signal_Limit/_minval: Value=KOUTP_FrEDUAvailBrkRgnTqV_flg_minval
      link override Signal_Override/_ovrdflg: Value=KOUTP_FrEDUAvailBrkRgnTqV_flg_ovrdflg
      link override Signal_Override/_ovrdval: Value=KOUTP_FrEDUAvailBrkRgnTqV_flg_ovrdval
  VTQD_FrEDUAvailBrkRgnTq_Nm_Inproc : FVT_lib/outp/OverrideAndLimit  SystemSampleTime=-1  VariantActivationTime=update diagram  Latency=0  AutoFrameSizeCalculation=off
      link override Signal_Limit/_maxval: Value=KOUTP_FrEDUAvailBrkRgnTq_Nm_maxval
      link override Signal_Limit/_minval: Value=KOUTP_FrEDUAvailBrkRgnTq_Nm_minval
      link override Signal_Override/_ovrdflg: Value=KOUTP_FrEDUAvailBrkRgnTq_Nm_ovrdflg
      link override Signal_Override/_ovrdval: Value=KOUTP_FrEDUAvailBrkRgnTq_Nm_ovrdval
  VTQD_FrEDURolRgnTq_Nm_Inproc : FVT_lib/outp/OverrideAndLimit  SystemSampleTime=-1  VariantActivationTime=update diagram  Latency=0  AutoFrameSizeCalculation=off
      link override Signal_Limit/_maxval: Value=KOUTP_FrEDURolRgnTq_Nm_maxval
      link override Signal_Limit/_minval: Value=KOUTP_FrEDURolRgnTq_Nm_minval
      link override Signal_Override/_ovrdflg: Value=KOUTP_FrEDURolRgnTq_Nm_ovrdflg
      link override Signal_Override/_ovrdval: Value=KOUTP_FrEDURolRgnTq_Nm_ovrdval
  VTQD_FrEDUSpdValid_flg_Inproc : FVT_lib/outp/OverrideAndLimit  SystemSampleTime=-1  VariantActivationTime=update diagram  Latency=0  AutoFrameSizeCalculation=off
      link override Signal_Limit/_maxval: Value=KOUTP_FrEDUSpdValid_flg_maxval
      link override Signal_Limit/_minval: Value=KOUTP_FrEDUSpdValid_flg_minval
      link override Signal_Override/_ovrdflg: Value=KOUTP_FrEDUSpdValid_flg_ovrdflg
      link override Signal_Override/_ovrdval: Value=KOUTP_FrEDUSpdValid_flg_ovrdval
  VTQD_FrEDUSpd_rpm_Inproc : FVT_lib/outp/OverrideAndLimit  SystemSampleTime=-1  VariantActivationTime=update diagram  Latency=0  AutoFrameSizeCalculation=off
      link override Signal_Limit/_maxval: Value=KOUTP_FrEDUSpd_rpm_maxval
      link override Signal_Limit/_minval: Value=KOUTP_FrEDUSpd_rpm_minval
      link override Signal_Override/_ovrdflg: Value=KOUTP_FrEDUSpd_rpm_ovrdflg
      link override Signal_Override/_ovrdval: Value=KOUTP_FrEDUSpd_rpm_ovrdval
  VTQD_FrIdcMax_A_Inproc : FVT_lib/outp/OverrideAndLimit  SystemSampleTime=-1  VariantActivationTime=update diagram  Latency=0  AutoFrameSizeCalculation=off
      link override Signal_Limit/_maxval: Value=KOUTP_FrIdcMax_A_maxval
      link override Signal_Limit/_minval: Value=KOUTP_FrIdcMax_A_minval
      link override Signal_Override/_ovrdflg: Value=KOUTP_FrIdcMax_A_ovrdflg
      link override Signal_Override/_ovrdval: Value=KOUTP_FrIdcMax_A_ovrdval
  VTQD_FrIdcMin_A_Inproc : FVT_lib/outp/OverrideAndLimit  SystemSampleTime=-1  VariantActivationTime=update diagram  Latency=0  AutoFrameSizeCalculation=off
      link override Signal_Limit/_maxval: Value=KOUTP_FrIdcMin_A_maxval
      link override Signal_Limit/_minval: Value=KOUTP_FrIdcMin_A_minval
      link override Signal_Override/_ovrdflg: Value=KOUTP_FrIdcMin_A_ovrdflg
      link override Signal_Override/_ovrdval: Value=KOUTP_FrIdcMin_A_ovrdval
  VTQD_FrRgnDecrSta_flg_Inproc : FVT_lib/outp/OverrideAndLimit  SystemSampleTime=-1  VariantActivationTime=update diagram  Latency=0  AutoFrameSizeCalculation=off
      link override Signal_Limit/_maxval: Value=KOUTP_FrRgnDecrSta_flg_maxval
      link override Signal_Limit/_minval: Value=KOUTP_FrRgnDecrSta_flg_minval
      link override Signal_Override/_ovrdflg: Value=KOUTP_FrRgnDecrSta_flg_ovrdflg
      link override Signal_Override/_ovrdval: Value=KOUTP_FrRgnDecrSta_flg_ovrdval
  VTQD_FrRgnPermSta_flg_Inproc : FVT_lib/outp/OverrideAndLimit  SystemSampleTime=-1  VariantActivationTime=update diagram  Latency=0  AutoFrameSizeCalculation=off
      link override Signal_Limit/_maxval: Value=KOUTP_FrRgnPermSta_flg_maxval
      link override Signal_Limit/_minval: Value=KOUTP_FrRgnPermSta_flg_minval
      link override Signal_Override/_ovrdflg: Value=KOUTP_FrRgnPermSta_flg_ovrdflg
      link override Signal_Override/_ovrdval: Value=KOUTP_FrRgnPermSta_flg_ovrdval
  VTQD_FrUdcMax_V_Inproc : FVT_lib/outp/OverrideAndLimit  SystemSampleTime=-1  VariantActivationTime=update diagram  Latency=0  AutoFrameSizeCalculation=off
      link override Signal_Limit/_maxval: Value=KOUTP_FrUdcMax_V_maxval
      link override Signal_Limit/_minval: Value=KOUTP_FrUdcMax_V_minval
      link override Signal_Override/_ovrdflg: Value=KOUTP_FrUdcMax_V_ovrdflg
      link override Signal_Override/_ovrdval: Value=KOUTP_FrUdcMax_V_ovrdval
  VTQD_FrUdcMin_V_Inproc : FVT_lib/outp/OverrideAndLimit  SystemSampleTime=-1  VariantActivationTime=update diagram  Latency=0  AutoFrameSizeCalculation=off
      link override Signal_Limit/_maxval: Value=KOUTP_FrUdcMin_V_maxval
      link override Signal_Limit/_minval: Value=KOUTP_FrUdcMin_V_minval
      link override Signal_Override/_ovrdflg: Value=KOUTP_FrUdcMin_V_ovrdflg
      link override Signal_Override/_ovrdval: Value=KOUTP_FrUdcMin_V_ovrdval
  VTQD_IVIPwrLockSta_enum_Inproc : FVT_lib/outp/OverrideAndLimit  SystemSampleTime=-1  VariantActivationTime=update diagram  Latency=0  AutoFrameSizeCalculation=off
      link override Signal_Limit/_maxval: Value=KOUTP_IVIPwrLockSta_enum_maxval
      link override Signal_Limit/_minval: Value=KOUTP_IVIPwrLockSta_enum_minval
      link override Signal_Override/_ovrdflg: Value=KOUTP_IVIPwrLockSta_enum_ovrdflg
      link override Signal_Override/_ovrdval: Value=KOUTP_IVIPwrLockSta_enum_ovrdval
  VTQD_OPDHoldLamp_flg_Inproc : FVT_lib/outp/OverrideAndLimit  SystemSampleTime=-1  VariantActivationTime=update diagram  Latency=0  AutoFrameSizeCalculation=off
      link override Signal_Limit/_maxval: Value=KOUTP_OPDHoldLamp_flg_maxval
      link override Signal_Limit/_minval: Value=KOUTP_OPDHoldLamp_flg_minval
      link override Signal_Override/_ovrdflg: Value=KOUTP_OPDHoldLamp_flg_ovrdflg
      link override Signal_Override/_ovrdval: Value=KOUTP_OPDHoldLamp_flg_ovrdval
  VTQD_PButtonSta_enum_Inproc : FVT_lib/outp/OverrideAndLimit  SystemSampleTime=-1  VariantActivationTime=update diagram  Latency=0  AutoFrameSizeCalculation=off
      link override Signal_Limit/_maxval: Value=KOUTP_PButtonSta_enum_maxval
      link override Signal_Limit/_minval: Value=KOUTP_PButtonSta_enum_minval
      link override Signal_Override/_ovrdflg: Value=KOUTP_PButtonSta_enum_ovrdflg
      link override Signal_Override/_ovrdval: Value=KOUTP_PButtonSta_enum_ovrdval
  VTQD_PTCSPermSta_flg_Inproc : FVT_lib/outp/OverrideAndLimit  SystemSampleTime=-1  VariantActivationTime=update diagram  Latency=0  AutoFrameSizeCalculation=off
      link override Signal_Limit/_maxval: Value=KOUTP_PTCSPermSta_flg_maxval
      link override Signal_Limit/_minval: Value=KOUTP_PTCSPermSta_flg_minval
      link override Signal_Override/_ovrdflg: Value=KOUTP_PTCSPermSta_flg_ovrdflg
      link override Signal_Override/_ovrdval: Value=KOUTP_PTCSPermSta_flg_ovrdval
  VTQD_ParkRequest_flg_Inproc : FVT_lib/outp/OverrideAndLimit  SystemSampleTime=-1  VariantActivationTime=update diagram  Latency=0  AutoFrameSizeCalculation=off
      link override Signal_Limit/_maxval: Value=KOUTP_ParkRequest_flg_maxval
      link override Signal_Limit/_minval: Value=KOUTP_ParkRequest_flg_minval
      link override Signal_Override/_ovrdflg: Value=KOUTP_ParkRequest_flg_ovrdflg
      link override Signal_Override/_ovrdval: Value=KOUTP_ParkRequest_flg_ovrdval
  VTQD_ReBrakeLPReq_flg_Inproc : FVT_lib/outp/OverrideAndLimit  SystemSampleTime=-1  VariantActivationTime=update diagram  Latency=0  AutoFrameSizeCalculation=off
      link override Signal_Limit/_maxval: Value=KOUTP_ReBrakeLPReq_flg_maxval
      link override Signal_Limit/_minval: Value=KOUTP_ReBrakeLPReq_flg_minval
      link override Signal_Override/_ovrdflg: Value=KOUTP_ReBrakeLPReq_flg_ovrdflg
      link override Signal_Override/_ovrdval: Value=KOUTP_ReBrakeLPReq_flg_ovrdval
  VTQD_RegenLimIndSta_flg_Inproc : FVT_lib/outp/OverrideAndLimit  SystemSampleTime=-1  VariantActivationTime=update diagram  Latency=0  AutoFrameSizeCalculation=off
      link override Signal_Limit/_maxval: Value=KOUTP_RegenLimIndSta_flg_maxval
      link override Signal_Limit/_minval: Value=KOUTP_RegenLimIndSta_flg_minval
      link override Signal_Override/_ovrdflg: Value=KOUTP_RegenLimIndSta_flg_ovrdflg
      link override Signal_Override/_ovrdval: Value=KOUTP_RegenLimIndSta_flg_ovrdval
  VTQD_RgnAbnorSta_flg_Inproc : FVT_lib/outp/OverrideAndLimit  SystemSampleTime=-1  VariantActivationTime=update diagram  Latency=0  AutoFrameSizeCalculation=off
      link override Signal_Limit/_maxval: Value=KOUTP_RgnAbnorSta_flg_maxval
      link override Signal_Limit/_minval: Value=KOUTP_RgnAbnorSta_flg_minval
      link override Signal_Override/_ovrdflg: Value=KOUTP_RgnAbnorSta_flg_ovrdflg
      link override Signal_Override/_ovrdval: Value=KOUTP_RgnAbnorSta_flg_ovrdval
  VTQD_RrActvDmpDisabReq_flg_Inproc : FVT_lib/outp/OverrideAndLimit  SystemSampleTime=-1  VariantActivationTime=update diagram  Latency=0  AutoFrameSizeCalculation=off
      link override Signal_Limit/_maxval: Value=KOUTP_RrActvDmpDisabReq_flg_maxval
      link override Signal_Limit/_minval: Value=KOUTP_RrActvDmpDisabReq_flg_minval
      link override Signal_Override/_ovrdflg: Value=KOUTP_RrActvDmpDisabReq_flg_ovrdflg
      link override Signal_Override/_ovrdval: Value=KOUTP_RrActvDmpDisabReq_flg_ovrdval
  VTQD_RrEDUActTq_Nm_Inproc : FVT_lib/outp/OverrideAndLimit  SystemSampleTime=-1  VariantActivationTime=update diagram  Latency=0  AutoFrameSizeCalculation=off
      link override Signal_Limit/_maxval: Value=KOUTP_RrEDUActTq_Nm_maxval
      link override Signal_Limit/_minval: Value=KOUTP_RrEDUActTq_Nm_minval
      link override Signal_Override/_ovrdflg: Value=KOUTP_RrEDUActTq_Nm_ovrdflg
      link override Signal_Override/_ovrdval: Value=KOUTP_RrEDUActTq_Nm_ovrdval
  VTQD_RrEDUAvailBrkRgnTqV_flg_Inproc : FVT_lib/outp/OverrideAndLimit  SystemSampleTime=-1  VariantActivationTime=update diagram  Latency=0  AutoFrameSizeCalculation=off
      link override Signal_Limit/_maxval: Value=KOUTP_RrEDUAvailBrkRgnTqV_flg_maxval
      link override Signal_Limit/_minval: Value=KOUTP_RrEDUAvailBrkRgnTqV_flg_minval
      link override Signal_Override/_ovrdflg: Value=KOUTP_RrEDUAvailBrkRgnTqV_flg_ovrdflg
      link override Signal_Override/_ovrdval: Value=KOUTP_RrEDUAvailBrkRgnTqV_flg_ovrdval
  VTQD_RrEDUAvailBrkRgnTq_Nm_Inproc : FVT_lib/outp/OverrideAndLimit  SystemSampleTime=-1  VariantActivationTime=update diagram  Latency=0  AutoFrameSizeCalculation=off
      link override Signal_Limit/_maxval: Value=KOUTP_RrEDUAvailBrkRgnTq_Nm_maxval
      link override Signal_Limit/_minval: Value=KOUTP_RrEDUAvailBrkRgnTq_Nm_minval
      link override Signal_Override/_ovrdflg: Value=KOUTP_RrEDUAvailBrkRgnTq_Nm_ovrdflg
      link override Signal_Override/_ovrdval: Value=KOUTP_RrEDUAvailBrkRgnTq_Nm_ovrdval
  VTQD_RrEDURolRgnTq_Nm_Inproc : FVT_lib/outp/OverrideAndLimit  SystemSampleTime=-1  VariantActivationTime=update diagram  Latency=0  AutoFrameSizeCalculation=off
      link override Signal_Limit/_maxval: Value=KOUTP_RrEDURolRgnTq_Nm_maxval
      link override Signal_Limit/_minval: Value=KOUTP_RrEDURolRgnTq_Nm_minval
      link override Signal_Override/_ovrdflg: Value=KOUTP_RrEDURolRgnTq_Nm_ovrdflg
      link override Signal_Override/_ovrdval: Value=KOUTP_RrEDURolRgnTq_Nm_ovrdval
  VTQD_RrEDUSpdValid_flg_Inproc : FVT_lib/outp/OverrideAndLimit  SystemSampleTime=-1  VariantActivationTime=update diagram  Latency=0  AutoFrameSizeCalculation=off
      link override Signal_Limit/_maxval: Value=KOUTP_RrEDUSpdValid_flg_maxval
      link override Signal_Limit/_minval: Value=KOUTP_RrEDUSpdValid_flg_minval
      link override Signal_Override/_ovrdflg: Value=KOUTP_RrEDUSpdValid_flg_ovrdflg
      link override Signal_Override/_ovrdval: Value=KOUTP_RrEDUSpdValid_flg_ovrdval
  VTQD_RrEDUSpd_rpm_Inproc : FVT_lib/outp/OverrideAndLimit  SystemSampleTime=-1  VariantActivationTime=update diagram  Latency=0  AutoFrameSizeCalculation=off
      link override Signal_Limit/_maxval: Value=KOUTP_RrEDUSpd_rpm_maxval
      link override Signal_Limit/_minval: Value=KOUTP_RrEDUSpd_rpm_minval
      link override Signal_Override/_ovrdflg: Value=KOUTP_RrEDUSpd_rpm_ovrdflg
      link override Signal_Override/_ovrdval: Value=KOUTP_RrEDUSpd_rpm_ovrdval
  VTQD_RrIdcMax_A_Inproc : FVT_lib/outp/OverrideAndLimit  SystemSampleTime=-1  VariantActivationTime=update diagram  Latency=0  AutoFrameSizeCalculation=off
      link override Signal_Limit/_maxval: Value=KOUTP_RrIdcMax_A_maxval
      link override Signal_Limit/_minval: Value=KOUTP_RrIdcMax_A_minval
      link override Signal_Override/_ovrdflg: Value=KOUTP_RrIdcMax_A_ovrdflg
      link override Signal_Override/_ovrdval: Value=KOUTP_RrIdcMax_A_ovrdval
  VTQD_RrIdcMin_A_Inproc : FVT_lib/outp/OverrideAndLimit  SystemSampleTime=-1  VariantActivationTime=update diagram  Latency=0  AutoFrameSizeCalculation=off
      link override Signal_Limit/_maxval: Value=KOUTP_RrIdcMin_A_maxval
      link override Signal_Limit/_minval: Value=KOUTP_RrIdcMin_A_minval
      link override Signal_Override/_ovrdflg: Value=KOUTP_RrIdcMin_A_ovrdflg
      link override Signal_Override/_ovrdval: Value=KOUTP_RrIdcMin_A_ovrdval
  VTQD_RrRgnDecrSta_flg_Inproc : FVT_lib/outp/OverrideAndLimit  SystemSampleTime=-1  VariantActivationTime=update diagram  Latency=0  AutoFrameSizeCalculation=off
      link override Signal_Limit/_maxval: Value=KOUTP_RrRgnDecrSta_flg_maxval
      link override Signal_Limit/_minval: Value=KOUTP_RrRgnDecrSta_flg_minval
      link override Signal_Override/_ovrdflg: Value=KOUTP_RrRgnDecrSta_flg_ovrdflg
      link override Signal_Override/_ovrdval: Value=KOUTP_RrRgnDecrSta_flg_ovrdval
  VTQD_RrRgnPermSta_flg_Inproc : FVT_lib/outp/OverrideAndLimit  SystemSampleTime=-1  VariantActivationTime=update diagram  Latency=0  AutoFrameSizeCalculation=off
      link override Signal_Limit/_maxval: Value=KOUTP_RrRgnPermSta_flg_maxval
      link override Signal_Limit/_minval: Value=KOUTP_RrRgnPermSta_flg_minval
      link override Signal_Override/_ovrdflg: Value=KOUTP_RrRgnPermSta_flg_ovrdflg
      link override Signal_Override/_ovrdval: Value=KOUTP_RrRgnPermSta_flg_ovrdval
  VTQD_RrUdcMax_V_Inproc : FVT_lib/outp/OverrideAndLimit  SystemSampleTime=-1  VariantActivationTime=update diagram  Latency=0  AutoFrameSizeCalculation=off
      link override Signal_Limit/_maxval: Value=KOUTP_RrUdcMax_V_maxval
      link override Signal_Limit/_minval: Value=KOUTP_RrUdcMax_V_minval
      link override Signal_Override/_ovrdflg: Value=KOUTP_RrUdcMax_V_ovrdflg
      link override Signal_Override/_ovrdval: Value=KOUTP_RrUdcMax_V_ovrdval
  VTQD_RrUdcMin_V_Inproc : FVT_lib/outp/OverrideAndLimit  SystemSampleTime=-1  VariantActivationTime=update diagram  Latency=0  AutoFrameSizeCalculation=off
      link override Signal_Limit/_maxval: Value=KOUTP_RrUdcMin_V_maxval
      link override Signal_Limit/_minval: Value=KOUTP_RrUdcMin_V_minval
      link override Signal_Override/_ovrdflg: Value=KOUTP_RrUdcMin_V_ovrdflg
      link override Signal_Override/_ovrdval: Value=KOUTP_RrUdcMin_V_ovrdval
  VTQD_SaveRegenMode_enum_Inproc : FVT_lib/outp/OverrideAndLimit  SystemSampleTime=-1  VariantActivationTime=update diagram  Latency=0  AutoFrameSizeCalculation=off
      link override Signal_Limit/_maxval: Value=KOUTP_SaveRegenMode_enum_maxval
      link override Signal_Limit/_minval: Value=KOUTP_SaveRegenMode_enum_minval
      link override Signal_Override/_ovrdflg: Value=KOUTP_SaveRegenMode_enum_ovrdflg
      link override Signal_Override/_ovrdval: Value=KOUTP_SaveRegenMode_enum_ovrdval
  VTQD_SetSpdLimWarn_flg_Inproc : FVT_lib/outp/OverrideAndLimit  SystemSampleTime=-1  VariantActivationTime=update diagram  Latency=0  AutoFrameSizeCalculation=off
      link override Signal_Limit/_maxval: Value=KOUTP_SetSpdLimWarn_flg_maxval
      link override Signal_Limit/_minval: Value=KOUTP_SetSpdLimWarn_flg_minval
      link override Signal_Override/_ovrdflg: Value=KOUTP_SetSpdLimWarn_flg_ovrdflg
      link override Signal_Override/_ovrdval: Value=KOUTP_SetSpdLimWarn_flg_ovrdval
  VTQD_SetSpd_kph_Inproc : FVT_lib/outp/OverrideAndLimit  SystemSampleTime=-1  VariantActivationTime=update diagram  Latency=0  AutoFrameSizeCalculation=off
      link override Signal_Limit/_maxval: Value=KOUTP_SetSpd_kph_maxval
      link override Signal_Limit/_minval: Value=KOUTP_SetSpd_kph_minval
      link override Signal_Override/_ovrdflg: Value=KOUTP_SetSpd_kph_ovrdflg
      link override Signal_Override/_ovrdval: Value=KOUTP_SetSpd_kph_ovrdval
  VTQD_ShiftGearPosn_enum_Inproc : FVT_lib/outp/OverrideAndLimit  SystemSampleTime=-1  VariantActivationTime=update diagram  Latency=0  AutoFrameSizeCalculation=off
      link override Signal_Limit/_maxval: Value=KOUTP_ShiftGearPosn_enum_maxval
      link override Signal_Limit/_minval: Value=KOUTP_ShiftGearPosn_enum_minval
      link override Signal_Override/_ovrdflg: Value=KOUTP_ShiftGearPosn_enum_ovrdflg
      link override Signal_Override/_ovrdval: Value=KOUTP_ShiftGearPosn_enum_ovrdval
  VTQD_SpdCtrlMode_enum_Inproc : FVT_lib/outp/OverrideAndLimit  SystemSampleTime=-1  VariantActivationTime=update diagram  Latency=0  AutoFrameSizeCalculation=off
      link override Signal_Limit/_maxval: Value=KOUTP_SpdCtrlMode_enum_maxval
      link override Signal_Limit/_minval: Value=KOUTP_SpdCtrlMode_enum_minval
      link override Signal_Override/_ovrdflg: Value=KOUTP_SpdCtrlMode_enum_ovrdflg
      link override Signal_Override/_ovrdval: Value=KOUTP_SpdCtrlMode_enum_ovrdval
  VTQD_SpdCtrlSta_flg_Inproc : FVT_lib/outp/OverrideAndLimit  SystemSampleTime=-1  VariantActivationTime=update diagram  Latency=0  AutoFrameSizeCalculation=off
      link override Signal_Limit/_maxval: Value=KOUTP_SpdCtrlSta_flg_maxval
      link override Signal_Limit/_minval: Value=KOUTP_SpdCtrlSta_flg_minval
      link override Signal_Override/_ovrdflg: Value=KOUTP_SpdCtrlSta_flg_ovrdflg
      link override Signal_Override/_ovrdval: Value=KOUTP_SpdCtrlSta_flg_ovrdval
  VTQD_TqSourceFr_enum_Inproc : FVT_lib/outp/OverrideAndLimit  SystemSampleTime=-1  VariantActivationTime=update diagram  Latency=0  AutoFrameSizeCalculation=off
      link override Signal_Limit/_maxval: Value=KOUTP_TqSourceFr_enum_maxval
      link override Signal_Limit/_minval: Value=KOUTP_TqSourceFr_enum_minval
      link override Signal_Override/_ovrdflg: Value=KOUTP_TqSourceFr_enum_ovrdflg
      link override Signal_Override/_ovrdval: Value=KOUTP_TqSourceFr_enum_ovrdval
  VTQD_TqSourceRr_enum_Inproc : FVT_lib/outp/OverrideAndLimit  SystemSampleTime=-1  VariantActivationTime=update diagram  Latency=0  AutoFrameSizeCalculation=off
      link override Signal_Limit/_maxval: Value=KOUTP_TqSourceRr_enum_maxval
      link override Signal_Limit/_minval: Value=KOUTP_TqSourceRr_enum_minval
      link override Signal_Override/_ovrdflg: Value=KOUTP_TqSourceRr_enum_ovrdflg
      link override Signal_Override/_ovrdval: Value=KOUTP_TqSourceRr_enum_ovrdval
  VTQD_VehActSpd_kph_Inproc : FVT_lib/outp/OverrideAndLimit  SystemSampleTime=-1  VariantActivationTime=update diagram  Latency=0  AutoFrameSizeCalculation=off
      link override Signal_Limit/_maxval: Value=KOUTP_VehActSpd_kph_maxval
      link override Signal_Limit/_minval: Value=KOUTP_VehActSpd_kph_minval
      link override Signal_Override/_ovrdflg: Value=KOUTP_VehActSpd_kph_ovrdflg
      link override Signal_Override/_ovrdval: Value=KOUTP_VehActSpd_kph_ovrdval
  VTQR_FrTMTqReq_Nm_Inproc : FVT_lib/outp/OverrideAndLimit  SystemSampleTime=-1  VariantActivationTime=update diagram  Latency=0  AutoFrameSizeCalculation=off
      link override Signal_Limit/_maxval: Value=KOUTP_FrTMTqReq_Nm_maxval
      link override Signal_Limit/_minval: Value=KOUTP_FrTMTqReq_Nm_minval
      link override Signal_Override/_ovrdflg: Value=KOUTP_FrTMTqReq_Nm_ovrdflg
      link override Signal_Override/_ovrdval: Value=KOUTP_FrTMTqReq_Nm_ovrdval
  VTQR_RrTMTqReq_Nm_Inproc : FVT_lib/outp/OverrideAndLimit  SystemSampleTime=-1  VariantActivationTime=update diagram  Latency=0  AutoFrameSizeCalculation=off
      link override Signal_Limit/_maxval: Value=KOUTP_RrTMTqReq_Nm_maxval
      link override Signal_Limit/_minval: Value=KOUTP_RrTMTqReq_Nm_minval
      link override Signal_Override/_ovrdflg: Value=KOUTP_RrTMTqReq_Nm_ovrdflg
      link override Signal_Override/_ovrdval: Value=KOUTP_RrTMTqReq_Nm_ovrdval
  VV2L_HVPO120VGrpALDSt_enum_Inproc : FVT_lib/outp/OverrideAndLimit  SystemSampleTime=-1  VariantActivationTime=update diagram  Latency=0  AutoFrameSizeCalculation=off
      link override Signal_Limit/_maxval: Value=KOUTP_HVPO120VGrpALDSt_enum_maxval
      link override Signal_Limit/_minval: Value=KOUTP_HVPO120VGrpALDSt_enum_minval
      link override Signal_Override/_ovrdflg: Value=KOUTP_HVPO120VGrpALDSt_enum_ovrdflg
      link override Signal_Override/_ovrdval: Value=KOUTP_HVPO120VGrpALDSt_enum_ovrdval
  VV2L_HVPO120VGrpBLDSt_enum_Inproc : FVT_lib/outp/OverrideAndLimit  SystemSampleTime=-1  VariantActivationTime=update diagram  Latency=0  AutoFrameSizeCalculation=off
      link override Signal_Limit/_maxval: Value=KOUTP_HVPO120VGrpBLDSt_enum_maxval
      link override Signal_Limit/_minval: Value=KOUTP_HVPO120VGrpBLDSt_enum_minval
      link override Signal_Override/_ovrdflg: Value=KOUTP_HVPO120VGrpBLDSt_enum_ovrdflg
      link override Signal_Override/_ovrdval: Value=KOUTP_HVPO120VGrpBLDSt_enum_ovrdval
  VV2L_ReqOBCExtrV2LEna_enum_Inproc : FVT_lib/outp/OverrideAndLimit  SystemSampleTime=-1  VariantActivationTime=update diagram  Latency=0  AutoFrameSizeCalculation=off
      link override Signal_Limit/_maxval: Value=KOUTP_ReqOBCExtrV2LEna_enum_maxval
      link override Signal_Limit/_minval: Value=KOUTP_ReqOBCExtrV2LEna_enum_minval
      link override Signal_Override/_ovrdflg: Value=KOUTP_ReqOBCExtrV2LEna_enum_ovrdflg
      link override Signal_Override/_ovrdval: Value=KOUTP_ReqOBCExtrV2LEna_enum_ovrdval
  VV2L_ReqOBCIntrV2LEna_enum_Inproc : FVT_lib/outp/OverrideAndLimit  SystemSampleTime=-1  VariantActivationTime=update diagram  Latency=0  AutoFrameSizeCalculation=off
      link override Signal_Limit/_maxval: Value=KOUTP_ReqOBCIntrV2LEna_enum_maxval
      link override Signal_Limit/_minval: Value=KOUTP_ReqOBCIntrV2LEna_enum_minval
      link override Signal_Override/_ovrdflg: Value=KOUTP_ReqOBCIntrV2LEna_enum_ovrdflg
      link override Signal_Override/_ovrdval: Value=KOUTP_ReqOBCIntrV2LEna_enum_ovrdval
  VV2L_ReqOBCV2LEna_enum_Inproc : FVT_lib/outp/OverrideAndLimit  SystemSampleTime=-1  VariantActivationTime=update diagram  Latency=0  AutoFrameSizeCalculation=off
      link override Signal_Limit/_maxval: Value=KOUTP_ReqOBCV2LEna_enum_maxval
      link override Signal_Limit/_minval: Value=KOUTP_ReqOBCV2LEna_enum_minval
      link override Signal_Override/_ovrdflg: Value=KOUTP_ReqOBCV2LEna_enum_ovrdflg
      link override Signal_Override/_ovrdval: Value=KOUTP_ReqOBCV2LEna_enum_ovrdval
  VV2L_ReqV2LIVIDisChrg_enum_Inproc : FVT_lib/outp/OverrideAndLimit  SystemSampleTime=-1  VariantActivationTime=update diagram  Latency=0  AutoFrameSizeCalculation=off
      link override Signal_Limit/_maxval: Value=KOUTP_ReqV2LIVIDisChrg_enum_maxval
      link override Signal_Limit/_minval: Value=KOUTP_ReqV2LIVIDisChrg_enum_minval
      link override Signal_Override/_ovrdflg: Value=KOUTP_ReqV2LIVIDisChrg_enum_ovrdflg
      link override Signal_Override/_ovrdval: Value=KOUTP_ReqV2LIVIDisChrg_enum_ovrdval
  VV2L_ReqV2LIVIPopup_enum_Inproc : FVT_lib/outp/OverrideAndLimit  SystemSampleTime=-1  VariantActivationTime=update diagram  Latency=0  AutoFrameSizeCalculation=off
      link override Signal_Limit/_maxval: Value=KOUTP_ReqV2LIVIPopup_enum_maxval
      link override Signal_Limit/_minval: Value=KOUTP_ReqV2LIVIPopup_enum_minval
      link override Signal_Override/_ovrdflg: Value=KOUTP_ReqV2LIVIPopup_enum_ovrdflg
      link override Signal_Override/_ovrdval: Value=KOUTP_ReqV2LIVIPopup_enum_ovrdval
  VVMC_ACCComfortBandLower_mps2_Inproc : FVT_lib/outp/OverrideAndLimit  SystemSampleTime=-1  VariantActivationTime=update diagram  Latency=0  AutoFrameSizeCalculation=off
      link override Signal_Limit/_maxval: Value=KOUTP_ACCComfortBandLower_mps2_maxval
      link override Signal_Limit/_minval: Value=KOUTP_ACCComfortBandLower_mps2_minval
      link override Signal_Override/_ovrdflg: Value=KOUTP_ACCComfortBandLower_mps2_ovrdflg
      link override Signal_Override/_ovrdval: Value=KOUTP_ACCComfortBandLower_mps2_ovrdval
  VVMC_ACCComfortBandUpper_mps2_Inproc : FVT_lib/outp/OverrideAndLimit  SystemSampleTime=-1  VariantActivationTime=update diagram  Latency=0  AutoFrameSizeCalculation=off
      link override Signal_Limit/_maxval: Value=KOUTP_ACCComfortBandUpper_mps2_maxval
      link override Signal_Limit/_minval: Value=KOUTP_ACCComfortBandUpper_mps2_minval
      link override Signal_Override/_ovrdflg: Value=KOUTP_ACCComfortBandUpper_mps2_ovrdflg
      link override Signal_Override/_ovrdval: Value=KOUTP_ACCComfortBandUpper_mps2_ovrdval
  VVMC_ACCCtrlAvail_flg_Inproc : FVT_lib/outp/OverrideAndLimit  SystemSampleTime=-1  VariantActivationTime=update diagram  Latency=0  AutoFrameSizeCalculation=off
      link override Signal_Limit/_maxval: Value=KOUTP_ACCCtrlAvail_flg_maxval
      link override Signal_Limit/_minval: Value=KOUTP_ACCCtrlAvail_flg_minval
      link override Signal_Override/_ovrdflg: Value=KOUTP_ACCCtrlAvail_flg_ovrdflg
      link override Signal_Override/_ovrdval: Value=KOUTP_ACCCtrlAvail_flg_ovrdval
  VVMC_ACCJerkLowerLimit_mps3_Inproc : FVT_lib/outp/OverrideAndLimit  SystemSampleTime=-1  VariantActivationTime=update diagram  Latency=0  AutoFrameSizeCalculation=off
      link override Signal_Limit/_maxval: Value=KOUTP_ACCJerkLowerLimit_mps3_maxval
      link override Signal_Limit/_minval: Value=KOUTP_ACCJerkLowerLimit_mps3_minval
      link override Signal_Override/_ovrdflg: Value=KOUTP_ACCJerkLowerLimit_mps3_ovrdflg
      link override Signal_Override/_ovrdval: Value=KOUTP_ACCJerkLowerLimit_mps3_ovrdval
  VVMC_ACCJerkUpperLimit_mps3_Inproc : FVT_lib/outp/OverrideAndLimit  SystemSampleTime=-1  VariantActivationTime=update diagram  Latency=0  AutoFrameSizeCalculation=off
      link override Signal_Limit/_maxval: Value=KOUTP_ACCJerkUpperLimit_mps3_maxval
      link override Signal_Limit/_minval: Value=KOUTP_ACCJerkUpperLimit_mps3_minval
      link override Signal_Override/_ovrdflg: Value=KOUTP_ACCJerkUpperLimit_mps3_ovrdflg
      link override Signal_Override/_ovrdval: Value=KOUTP_ACCJerkUpperLimit_mps3_ovrdval
  VVMC_ACCObjDist_m_Inproc : FVT_lib/outp/OverrideAndLimit  SystemSampleTime=-1  VariantActivationTime=update diagram  Latency=0  AutoFrameSizeCalculation=off
      link override Signal_Limit/_maxval: Value=KOUTP_ACCObjDist_m_maxval
      link override Signal_Limit/_minval: Value=KOUTP_ACCObjDist_m_minval
      link override Signal_Override/_ovrdflg: Value=KOUTP_ACCObjDist_m_ovrdflg
      link override Signal_Override/_ovrdval: Value=KOUTP_ACCObjDist_m_ovrdval
  VVMC_ACCObjDstLvl_enum_Inproc : FVT_lib/outp/OverrideAndLimit  SystemSampleTime=-1  VariantActivationTime=update diagram  Latency=0  AutoFrameSizeCalculation=off
      link override Signal_Limit/_maxval: Value=KOUTP_ACCObjDstLvl_enum_maxval
      link override Signal_Limit/_minval: Value=KOUTP_ACCObjDstLvl_enum_minval
      link override Signal_Override/_ovrdflg: Value=KOUTP_ACCObjDstLvl_enum_ovrdflg
      link override Signal_Override/_ovrdval: Value=KOUTP_ACCObjDstLvl_enum_ovrdval
  VVMC_ACCObjRelSpd_mps_Inproc : FVT_lib/outp/OverrideAndLimit  SystemSampleTime=-1  VariantActivationTime=update diagram  Latency=0  AutoFrameSizeCalculation=off
      link override Signal_Limit/_maxval: Value=KOUTP_ACCObjRelSpd_mps_maxval
      link override Signal_Limit/_minval: Value=KOUTP_ACCObjRelSpd_mps_minval
      link override Signal_Override/_ovrdflg: Value=KOUTP_ACCObjRelSpd_mps_ovrdflg
      link override Signal_Override/_ovrdval: Value=KOUTP_ACCObjRelSpd_mps_ovrdval
  VVMC_ACCPedalOvrd_flg_Inproc : FVT_lib/outp/OverrideAndLimit  SystemSampleTime=-1  VariantActivationTime=update diagram  Latency=0  AutoFrameSizeCalculation=off
      link override Signal_Limit/_maxval: Value=KOUTP_ACCPedalOvrd_flg_maxval
      link override Signal_Limit/_minval: Value=KOUTP_ACCPedalOvrd_flg_minval
      link override Signal_Override/_ovrdflg: Value=KOUTP_ACCPedalOvrd_flg_ovrdflg
      link override Signal_Override/_ovrdval: Value=KOUTP_ACCPedalOvrd_flg_ovrdval
  VVMC_ACCRequiredAccel_mps2_Inproc : FVT_lib/outp/OverrideAndLimit  SystemSampleTime=-1  VariantActivationTime=update diagram  Latency=0  AutoFrameSizeCalculation=off
      link override Signal_Limit/_maxval: Value=KOUTP_ACCRequiredAccel_mps2_maxval
      link override Signal_Limit/_minval: Value=KOUTP_ACCRequiredAccel_mps2_minval
      link override Signal_Override/_ovrdflg: Value=KOUTP_ACCRequiredAccel_mps2_ovrdflg
      link override Signal_Override/_ovrdval: Value=KOUTP_ACCRequiredAccel_mps2_ovrdval
  VVMC_ACCTakeoverReq_flg_Inproc : FVT_lib/outp/OverrideAndLimit  SystemSampleTime=-1  VariantActivationTime=update diagram  Latency=0  AutoFrameSizeCalculation=off
      link override Signal_Limit/_maxval: Value=KOUTP_ACCTakeoverReq_flg_maxval
      link override Signal_Limit/_minval: Value=KOUTP_ACCTakeoverReq_flg_minval
      link override Signal_Override/_ovrdflg: Value=KOUTP_ACCTakeoverReq_flg_ovrdflg
      link override Signal_Override/_ovrdval: Value=KOUTP_ACCTakeoverReq_flg_ovrdval
  VVMC_ACCVehHoldReq_flg_Inproc : FVT_lib/outp/OverrideAndLimit  SystemSampleTime=-1  VariantActivationTime=update diagram  Latency=0  AutoFrameSizeCalculation=off
      link override Signal_Limit/_maxval: Value=KOUTP_ACCVehHoldReq_flg_maxval
      link override Signal_Limit/_minval: Value=KOUTP_ACCVehHoldReq_flg_minval
      link override Signal_Override/_ovrdflg: Value=KOUTP_ACCVehHoldReq_flg_ovrdflg
      link override Signal_Override/_ovrdval: Value=KOUTP_ACCVehHoldReq_flg_ovrdval
  VVMC_ADASACCSta_enum_Inproc : FVT_lib/outp/OverrideAndLimit  SystemSampleTime=-1  VariantActivationTime=update diagram  Latency=0  AutoFrameSizeCalculation=off
      link override Signal_Limit/_maxval: Value=KOUTP_ADASACCSta_enum_maxval
      link override Signal_Limit/_minval: Value=KOUTP_ADASACCSta_enum_minval
      link override Signal_Override/_ovrdflg: Value=KOUTP_ADASACCSta_enum_ovrdflg
      link override Signal_Override/_ovrdval: Value=KOUTP_ADASACCSta_enum_ovrdval
  VVMC_ADASAEBReq_enum_Inproc : FVT_lib/outp/OverrideAndLimit  SystemSampleTime=-1  VariantActivationTime=update diagram  Latency=0  AutoFrameSizeCalculation=off
      link override Signal_Limit/_maxval: Value=KOUTP_ADASAEBReq_enum_maxval
      link override Signal_Limit/_minval: Value=KOUTP_ADASAEBReq_enum_minval
      link override Signal_Override/_ovrdflg: Value=KOUTP_ADASAEBReq_enum_ovrdflg
      link override Signal_Override/_ovrdval: Value=KOUTP_ADASAEBReq_enum_ovrdval
  VVMC_ADASAEBSta_enum_Inproc : FVT_lib/outp/OverrideAndLimit  SystemSampleTime=-1  VariantActivationTime=update diagram  Latency=0  AutoFrameSizeCalculation=off
      link override Signal_Limit/_maxval: Value=KOUTP_ADASAEBSta_enum_maxval
      link override Signal_Limit/_minval: Value=KOUTP_ADASAEBSta_enum_minval
      link override Signal_Override/_ovrdflg: Value=KOUTP_ADASAEBSta_enum_ovrdflg
      link override Signal_Override/_ovrdval: Value=KOUTP_ADASAEBSta_enum_ovrdval
  VVMC_ADASCAMSpdLim_enum_Inproc : FVT_lib/outp/OverrideAndLimit  SystemSampleTime=-1  VariantActivationTime=update diagram  Latency=0  AutoFrameSizeCalculation=off
      link override Signal_Limit/_maxval: Value=KOUTP_ADASCAMSpdLim_enum_maxval
      link override Signal_Limit/_minval: Value=KOUTP_ADASCAMSpdLim_enum_minval
      link override Signal_Override/_ovrdflg: Value=KOUTP_ADASCAMSpdLim_enum_ovrdflg
      link override Signal_Override/_ovrdval: Value=KOUTP_ADASCAMSpdLim_enum_ovrdval
  VVMC_ADASDBSReq_enum_Inproc : FVT_lib/outp/OverrideAndLimit  SystemSampleTime=-1  VariantActivationTime=update diagram  Latency=0  AutoFrameSizeCalculation=off
      link override Signal_Limit/_maxval: Value=KOUTP_ADASDBSReq_enum_maxval
      link override Signal_Limit/_minval: Value=KOUTP_ADASDBSReq_enum_minval
      link override Signal_Override/_ovrdflg: Value=KOUTP_ADASDBSReq_enum_ovrdflg
      link override Signal_Override/_ovrdval: Value=KOUTP_ADASDBSReq_enum_ovrdval
  VVMC_ADASFCWMute_flg_Inproc : FVT_lib/outp/OverrideAndLimit  SystemSampleTime=-1  VariantActivationTime=update diagram  Latency=0  AutoFrameSizeCalculation=off
      link override Signal_Limit/_maxval: Value=KOUTP_ADASFCWMute_flg_maxval
      link override Signal_Limit/_minval: Value=KOUTP_ADASFCWMute_flg_minval
      link override Signal_Override/_ovrdflg: Value=KOUTP_ADASFCWMute_flg_ovrdflg
      link override Signal_Override/_ovrdval: Value=KOUTP_ADASFCWMute_flg_ovrdval
  VVMC_ADASFCWSta_enum_Inproc : FVT_lib/outp/OverrideAndLimit  SystemSampleTime=-1  VariantActivationTime=update diagram  Latency=0  AutoFrameSizeCalculation=off
      link override Signal_Limit/_maxval: Value=KOUTP_ADASFCWSta_enum_maxval
      link override Signal_Limit/_minval: Value=KOUTP_ADASFCWSta_enum_minval
      link override Signal_Override/_ovrdflg: Value=KOUTP_ADASFCWSta_enum_ovrdflg
      link override Signal_Override/_ovrdval: Value=KOUTP_ADASFCWSta_enum_ovrdval
  VVMC_ADASFaultSta_flg_Inproc : FVT_lib/outp/OverrideAndLimit  SystemSampleTime=-1  VariantActivationTime=update diagram  Latency=0  AutoFrameSizeCalculation=off
      link override Signal_Limit/_maxval: Value=KOUTP_ADASFaultSta_flg_maxval
      link override Signal_Limit/_minval: Value=KOUTP_ADASFaultSta_flg_minval
      link override Signal_Override/_ovrdflg: Value=KOUTP_ADASFaultSta_flg_ovrdflg
      link override Signal_Override/_ovrdval: Value=KOUTP_ADASFaultSta_flg_ovrdval
  VVMC_ADASFltWrnReq_flg_Inproc : FVT_lib/outp/OverrideAndLimit  SystemSampleTime=-1  VariantActivationTime=update diagram  Latency=0  AutoFrameSizeCalculation=off
      link override Signal_Limit/_maxval: Value=KOUTP_ADASFltWrnReq_flg_maxval
      link override Signal_Limit/_minval: Value=KOUTP_ADASFltWrnReq_flg_minval
      link override Signal_Override/_ovrdflg: Value=KOUTP_ADASFltWrnReq_flg_ovrdflg
      link override Signal_Override/_ovrdval: Value=KOUTP_ADASFltWrnReq_flg_ovrdval
  VVMC_ADASForceIdle_flg_Inproc : FVT_lib/outp/OverrideAndLimit  SystemSampleTime=-1  VariantActivationTime=update diagram  Latency=0  AutoFrameSizeCalculation=off
      link override Signal_Limit/_maxval: Value=KOUTP_ADASForceIdle_flg_maxval
      link override Signal_Limit/_minval: Value=KOUTP_ADASForceIdle_flg_minval
      link override Signal_Override/_ovrdflg: Value=KOUTP_ADASForceIdle_flg_ovrdflg
      link override Signal_Override/_ovrdval: Value=KOUTP_ADASForceIdle_flg_ovrdval
  VVMC_ADASISASta_enum_Inproc : FVT_lib/outp/OverrideAndLimit  SystemSampleTime=-1  VariantActivationTime=update diagram  Latency=0  AutoFrameSizeCalculation=off
      link override Signal_Limit/_maxval: Value=KOUTP_ADASISASta_enum_maxval
      link override Signal_Limit/_minval: Value=KOUTP_ADASISASta_enum_minval
      link override Signal_Override/_ovrdflg: Value=KOUTP_ADASISASta_enum_ovrdflg
      link override Signal_Override/_ovrdval: Value=KOUTP_ADASISASta_enum_ovrdval
  VVMC_ADASLDWMute_flg_Inproc : FVT_lib/outp/OverrideAndLimit  SystemSampleTime=-1  VariantActivationTime=update diagram  Latency=0  AutoFrameSizeCalculation=off
      link override Signal_Limit/_maxval: Value=KOUTP_ADASLDWMute_flg_maxval
      link override Signal_Limit/_minval: Value=KOUTP_ADASLDWMute_flg_minval
      link override Signal_Override/_ovrdflg: Value=KOUTP_ADASLDWMute_flg_ovrdflg
      link override Signal_Override/_ovrdval: Value=KOUTP_ADASLDWMute_flg_ovrdval
  VVMC_ADASLDWSta_enum_Inproc : FVT_lib/outp/OverrideAndLimit  SystemSampleTime=-1  VariantActivationTime=update diagram  Latency=0  AutoFrameSizeCalculation=off
      link override Signal_Limit/_maxval: Value=KOUTP_ADASLDWSta_enum_maxval
      link override Signal_Limit/_minval: Value=KOUTP_ADASLDWSta_enum_minval
      link override Signal_Override/_ovrdflg: Value=KOUTP_ADASLDWSta_enum_ovrdflg
      link override Signal_Override/_ovrdval: Value=KOUTP_ADASLDWSta_enum_ovrdval
  VVMC_ADASLFCHandsOffWarning_enum_Inproc : FVT_lib/outp/OverrideAndLimit  SystemSampleTime=-1  VariantActivationTime=update diagram  Latency=0  AutoFrameSizeCalculation=off
      link override Signal_Limit/_maxval: Value=KOUTP_ADASLFCHandsOffWarning_enum_maxval
      link override Signal_Limit/_minval: Value=KOUTP_ADASLFCHandsOffWarning_enum_minval
      link override Signal_Override/_ovrdflg: Value=KOUTP_ADASLFCHandsOffWarning_enum_ovrdflg
      link override Signal_Override/_ovrdval: Value=KOUTP_ADASLFCHandsOffWarning_enum_ovrdval
  VVMC_ADASLFCSta_enum_Inproc : FVT_lib/outp/OverrideAndLimit  SystemSampleTime=-1  VariantActivationTime=update diagram  Latency=0  AutoFrameSizeCalculation=off
      link override Signal_Limit/_maxval: Value=KOUTP_ADASLFCSta_enum_maxval
      link override Signal_Limit/_minval: Value=KOUTP_ADASLFCSta_enum_minval
      link override Signal_Override/_ovrdflg: Value=KOUTP_ADASLFCSta_enum_ovrdflg
      link override Signal_Override/_ovrdval: Value=KOUTP_ADASLFCSta_enum_ovrdval
  VVMC_ADASLFCWarnSound_enum_Inproc : FVT_lib/outp/OverrideAndLimit  SystemSampleTime=-1  VariantActivationTime=update diagram  Latency=0  AutoFrameSizeCalculation=off
      link override Signal_Limit/_maxval: Value=KOUTP_ADASLFCWarnSound_enum_maxval
      link override Signal_Limit/_minval: Value=KOUTP_ADASLFCWarnSound_enum_minval
      link override Signal_Override/_ovrdflg: Value=KOUTP_ADASLFCWarnSound_enum_ovrdflg
      link override Signal_Override/_ovrdval: Value=KOUTP_ADASLFCWarnSound_enum_ovrdval
  VVMC_ADASLKASta_enum_Inproc : FVT_lib/outp/OverrideAndLimit  SystemSampleTime=-1  VariantActivationTime=update diagram  Latency=0  AutoFrameSizeCalculation=off
      link override Signal_Limit/_maxval: Value=KOUTP_ADASLKASta_enum_maxval
      link override Signal_Limit/_minval: Value=KOUTP_ADASLKASta_enum_minval
      link override Signal_Override/_ovrdflg: Value=KOUTP_ADASLKASta_enum_ovrdflg
      link override Signal_Override/_ovrdval: Value=KOUTP_ADASLKASta_enum_ovrdval
  VVMC_ADASLaneModeL_enum_Inproc : FVT_lib/outp/OverrideAndLimit  SystemSampleTime=-1  VariantActivationTime=update diagram  Latency=0  AutoFrameSizeCalculation=off
      link override Signal_Limit/_maxval: Value=KOUTP_ADASLaneModeL_enum_maxval
      link override Signal_Limit/_minval: Value=KOUTP_ADASLaneModeL_enum_minval
      link override Signal_Override/_ovrdflg: Value=KOUTP_ADASLaneModeL_enum_ovrdflg
      link override Signal_Override/_ovrdval: Value=KOUTP_ADASLaneModeL_enum_ovrdval
  VVMC_ADASLaneModeR_enum_Inproc : FVT_lib/outp/OverrideAndLimit  SystemSampleTime=-1  VariantActivationTime=update diagram  Latency=0  AutoFrameSizeCalculation=off
      link override Signal_Limit/_maxval: Value=KOUTP_ADASLaneModeR_enum_maxval
      link override Signal_Limit/_minval: Value=KOUTP_ADASLaneModeR_enum_minval
      link override Signal_Override/_ovrdflg: Value=KOUTP_ADASLaneModeR_enum_ovrdflg
      link override Signal_Override/_ovrdval: Value=KOUTP_ADASLaneModeR_enum_ovrdval
  VVMC_ADASLanecurveL_raw32_Inproc : FVT_lib/outp/OverrideAndLimit  SystemSampleTime=-1  VariantActivationTime=update diagram  Latency=0  AutoFrameSizeCalculation=off
      link override Signal_Limit/_maxval: Value=KOUTP_ADASLanecurveL_raw32_maxval
      link override Signal_Limit/_minval: Value=KOUTP_ADASLanecurveL_raw32_minval
      link override Signal_Override/_ovrdflg: Value=KOUTP_ADASLanecurveL_raw32_ovrdflg
      link override Signal_Override/_ovrdval: Value=KOUTP_ADASLanecurveL_raw32_ovrdval
  VVMC_ADASLanecurveR_raw32_Inproc : FVT_lib/outp/OverrideAndLimit  SystemSampleTime=-1  VariantActivationTime=update diagram  Latency=0  AutoFrameSizeCalculation=off
      link override Signal_Limit/_maxval: Value=KOUTP_ADASLanecurveR_raw32_maxval
      link override Signal_Limit/_minval: Value=KOUTP_ADASLanecurveR_raw32_minval
      link override Signal_Override/_ovrdflg: Value=KOUTP_ADASLanecurveR_raw32_ovrdflg
      link override Signal_Override/_ovrdval: Value=KOUTP_ADASLanecurveR_raw32_ovrdval
  VVMC_ADASLanetypeL_enum_Inproc : FVT_lib/outp/OverrideAndLimit  SystemSampleTime=-1  VariantActivationTime=update diagram  Latency=0  AutoFrameSizeCalculation=off
      link override Signal_Limit/_maxval: Value=KOUTP_ADASLanetypeL_enum_maxval
      link override Signal_Limit/_minval: Value=KOUTP_ADASLanetypeL_enum_minval
      link override Signal_Override/_ovrdflg: Value=KOUTP_ADASLanetypeL_enum_ovrdflg
      link override Signal_Override/_ovrdval: Value=KOUTP_ADASLanetypeL_enum_ovrdval
  VVMC_ADASLanetypeR_enum_Inproc : FVT_lib/outp/OverrideAndLimit  SystemSampleTime=-1  VariantActivationTime=update diagram  Latency=0  AutoFrameSizeCalculation=off
      link override Signal_Limit/_maxval: Value=KOUTP_ADASLanetypeR_enum_maxval
      link override Signal_Limit/_minval: Value=KOUTP_ADASLanetypeR_enum_minval
      link override Signal_Override/_ovrdflg: Value=KOUTP_ADASLanetypeR_enum_ovrdflg
      link override Signal_Override/_ovrdval: Value=KOUTP_ADASLanetypeR_enum_ovrdval
  VVMC_ADASSLIFSpdLim_enum_Inproc : FVT_lib/outp/OverrideAndLimit  SystemSampleTime=-1  VariantActivationTime=update diagram  Latency=0  AutoFrameSizeCalculation=off
      link override Signal_Limit/_maxval: Value=KOUTP_ADASSLIFSpdLim_enum_maxval
      link override Signal_Limit/_minval: Value=KOUTP_ADASSLIFSpdLim_enum_minval
      link override Signal_Override/_ovrdflg: Value=KOUTP_ADASSLIFSpdLim_enum_ovrdflg
      link override Signal_Override/_ovrdval: Value=KOUTP_ADASSLIFSpdLim_enum_ovrdval
  VVMC_ADASSLIFSta_enum_Inproc : FVT_lib/outp/OverrideAndLimit  SystemSampleTime=-1  VariantActivationTime=update diagram  Latency=0  AutoFrameSizeCalculation=off
      link override Signal_Limit/_maxval: Value=KOUTP_ADASSLIFSta_enum_maxval
      link override Signal_Limit/_minval: Value=KOUTP_ADASSLIFSta_enum_minval
      link override Signal_Override/_ovrdflg: Value=KOUTP_ADASSLIFSta_enum_ovrdflg
      link override Signal_Override/_ovrdval: Value=KOUTP_ADASSLIFSta_enum_ovrdval
  VVMC_ADASShftPosnReqA_flg_Inproc : FVT_lib/outp/OverrideAndLimit  SystemSampleTime=-1  VariantActivationTime=update diagram  Latency=0  AutoFrameSizeCalculation=off
      link override Signal_Limit/_maxval: Value=KOUTP_ADASShftPosnReqA_flg_maxval
      link override Signal_Limit/_minval: Value=KOUTP_ADASShftPosnReqA_flg_minval
      link override Signal_Override/_ovrdflg: Value=KOUTP_ADASShftPosnReqA_flg_ovrdflg
      link override Signal_Override/_ovrdval: Value=KOUTP_ADASShftPosnReqA_flg_ovrdval
  VVMC_ADASShftPosnReq_enum_Inproc : FVT_lib/outp/OverrideAndLimit  SystemSampleTime=-1  VariantActivationTime=update diagram  Latency=0  AutoFrameSizeCalculation=off
      link override Signal_Limit/_maxval: Value=KOUTP_ADASShftPosnReq_enum_maxval
      link override Signal_Limit/_minval: Value=KOUTP_ADASShftPosnReq_enum_minval
      link override Signal_Override/_ovrdflg: Value=KOUTP_ADASShftPosnReq_enum_ovrdflg
      link override Signal_Override/_ovrdval: Value=KOUTP_ADASShftPosnReq_enum_ovrdval
  VVMC_ADASVehSpdLim_raw32_Inproc : FVT_lib/outp/OverrideAndLimit  SystemSampleTime=-1  VariantActivationTime=update diagram  Latency=0  AutoFrameSizeCalculation=off
      link override Signal_Limit/_maxval: Value=KOUTP_ADASVehSpdLim_raw32_maxval
      link override Signal_Limit/_minval: Value=KOUTP_ADASVehSpdLim_raw32_minval
      link override Signal_Override/_ovrdflg: Value=KOUTP_ADASVehSpdLim_raw32_ovrdflg
      link override Signal_Override/_ovrdval: Value=KOUTP_ADASVehSpdLim_raw32_ovrdval
  VVMC_ADASWarningMsg_enum_Inproc : FVT_lib/outp/OverrideAndLimit  SystemSampleTime=-1  VariantActivationTime=update diagram  Latency=0  AutoFrameSizeCalculation=off
      link override Signal_Limit/_maxval: Value=KOUTP_ADASWarningMsg_enum_maxval
      link override Signal_Limit/_minval: Value=KOUTP_ADASWarningMsg_enum_minval
      link override Signal_Override/_ovrdflg: Value=KOUTP_ADASWarningMsg_enum_ovrdflg
      link override Signal_Override/_ovrdval: Value=KOUTP_ADASWarningMsg_enum_ovrdval
  VVMC_AEBVehHoldReq_flg_Inproc : FVT_lib/outp/OverrideAndLimit  SystemSampleTime=-1  VariantActivationTime=update diagram  Latency=0  AutoFrameSizeCalculation=off
      link override Signal_Limit/_maxval: Value=KOUTP_AEBVehHoldReq_flg_maxval
      link override Signal_Limit/_minval: Value=KOUTP_AEBVehHoldReq_flg_minval
      link override Signal_Override/_ovrdflg: Value=KOUTP_AEBVehHoldReq_flg_ovrdflg
      link override Signal_Override/_ovrdval: Value=KOUTP_AEBVehHoldReq_flg_ovrdval
  VVMC_APSActive_flg_Inproc : FVT_lib/outp/OverrideAndLimit  SystemSampleTime=-1  VariantActivationTime=update diagram  Latency=0  AutoFrameSizeCalculation=off
      link override Signal_Limit/_maxval: Value=KOUTP_APSActive_flg_maxval
      link override Signal_Limit/_minval: Value=KOUTP_APSActive_flg_minval
      link override Signal_Override/_ovrdflg: Value=KOUTP_APSActive_flg_ovrdflg
      link override Signal_Override/_ovrdval: Value=KOUTP_APSActive_flg_ovrdval
  VVMC_APSCtrlAvail_flg_Inproc : FVT_lib/outp/OverrideAndLimit  SystemSampleTime=-1  VariantActivationTime=update diagram  Latency=0  AutoFrameSizeCalculation=off
      link override Signal_Limit/_maxval: Value=KOUTP_APSCtrlAvail_flg_maxval
      link override Signal_Limit/_minval: Value=KOUTP_APSCtrlAvail_flg_minval
      link override Signal_Override/_ovrdflg: Value=KOUTP_APSCtrlAvail_flg_ovrdflg
      link override Signal_Override/_ovrdval: Value=KOUTP_APSCtrlAvail_flg_ovrdval
  VVMC_APSDecReqA_flg_Inproc : FVT_lib/outp/OverrideAndLimit  SystemSampleTime=-1  VariantActivationTime=update diagram  Latency=0  AutoFrameSizeCalculation=off
      link override Signal_Limit/_maxval: Value=KOUTP_APSDecReqA_flg_maxval
      link override Signal_Limit/_minval: Value=KOUTP_APSDecReqA_flg_minval
      link override Signal_Override/_ovrdflg: Value=KOUTP_APSDecReqA_flg_ovrdflg
      link override Signal_Override/_ovrdval: Value=KOUTP_APSDecReqA_flg_ovrdval
  VVMC_APSDecReq_mps2_Inproc : FVT_lib/outp/OverrideAndLimit  SystemSampleTime=-1  VariantActivationTime=update diagram  Latency=0  AutoFrameSizeCalculation=off
      link override Signal_Limit/_maxval: Value=KOUTP_APSDecReq_mps2_maxval
      link override Signal_Limit/_minval: Value=KOUTP_APSDecReq_mps2_minval
      link override Signal_Override/_ovrdflg: Value=KOUTP_APSDecReq_mps2_ovrdflg
      link override Signal_Override/_ovrdval: Value=KOUTP_APSDecReq_mps2_ovrdval
  VVMC_APSReq_enum_Inproc : FVT_lib/outp/OverrideAndLimit  SystemSampleTime=-1  VariantActivationTime=update diagram  Latency=0  AutoFrameSizeCalculation=off
      link override Signal_Limit/_maxval: Value=KOUTP_APSReq_enum_maxval
      link override Signal_Limit/_minval: Value=KOUTP_APSReq_enum_minval
      link override Signal_Override/_ovrdflg: Value=KOUTP_APSReq_enum_ovrdflg
      link override Signal_Override/_ovrdval: Value=KOUTP_APSReq_enum_ovrdval
  VVMC_APSStaSys_enum_Inproc : FVT_lib/outp/OverrideAndLimit  SystemSampleTime=-1  VariantActivationTime=update diagram  Latency=0  AutoFrameSizeCalculation=off
      link override Signal_Limit/_maxval: Value=KOUTP_APSStaSys_enum_maxval
      link override Signal_Limit/_minval: Value=KOUTP_APSStaSys_enum_minval
      link override Signal_Override/_ovrdflg: Value=KOUTP_APSStaSys_enum_ovrdflg
      link override Signal_Override/_ovrdval: Value=KOUTP_APSStaSys_enum_ovrdval
  VVMC_AccCalcuPID_mps2_Inproc : FVT_lib/outp/OverrideAndLimit  SystemSampleTime=-1  VariantActivationTime=update diagram  Latency=0  AutoFrameSizeCalculation=off
      link override Signal_Limit/_maxval: Value=KOUTP_AccCalcuPID_mps2_maxval
      link override Signal_Limit/_minval: Value=KOUTP_AccCalcuPID_mps2_minval
      link override Signal_Override/_ovrdflg: Value=KOUTP_AccCalcuPID_mps2_ovrdflg
      link override Signal_Override/_ovrdval: Value=KOUTP_AccCalcuPID_mps2_ovrdval
  VVMC_ActACCRequiredAccel_mps2_Inproc : FVT_lib/outp/OverrideAndLimit  SystemSampleTime=-1  VariantActivationTime=update diagram  Latency=0  AutoFrameSizeCalculation=off
      link override Signal_Limit/_maxval: Value=KOUTP_ActACCRequiredAccel_mps2_maxval
      link override Signal_Limit/_minval: Value=KOUTP_ActACCRequiredAccel_mps2_minval
      link override Signal_Override/_ovrdflg: Value=KOUTP_ActACCRequiredAccel_mps2_ovrdflg
      link override Signal_Override/_ovrdval: Value=KOUTP_ActACCRequiredAccel_mps2_ovrdval
  VVMC_CAASActive_flg_Inproc : FVT_lib/outp/OverrideAndLimit  SystemSampleTime=-1  VariantActivationTime=update diagram  Latency=0  AutoFrameSizeCalculation=off
      link override Signal_Limit/_maxval: Value=KOUTP_CAASActive_flg_maxval
      link override Signal_Limit/_minval: Value=KOUTP_CAASActive_flg_minval
      link override Signal_Override/_ovrdflg: Value=KOUTP_CAASActive_flg_ovrdflg
      link override Signal_Override/_ovrdval: Value=KOUTP_CAASActive_flg_ovrdval
  VVMC_CAASCtrlAvail_flg_Inproc : FVT_lib/outp/OverrideAndLimit  SystemSampleTime=-1  VariantActivationTime=update diagram  Latency=0  AutoFrameSizeCalculation=off
      link override Signal_Limit/_maxval: Value=KOUTP_CAASCtrlAvail_flg_maxval
      link override Signal_Limit/_minval: Value=KOUTP_CAASCtrlAvail_flg_minval
      link override Signal_Override/_ovrdflg: Value=KOUTP_CAASCtrlAvail_flg_ovrdflg
      link override Signal_Override/_ovrdval: Value=KOUTP_CAASCtrlAvail_flg_ovrdval
  VVMC_CCCtrlSta_enum_Inproc : FVT_lib/outp/OverrideAndLimit  SystemSampleTime=-1  VariantActivationTime=update diagram  Latency=0  AutoFrameSizeCalculation=off
      link override Signal_Limit/_maxval: Value=KOUTP_CCCtrlSta_enum_maxval
      link override Signal_Limit/_minval: Value=KOUTP_CCCtrlSta_enum_minval
      link override Signal_Override/_ovrdflg: Value=KOUTP_CCCtrlSta_enum_ovrdflg
      link override Signal_Override/_ovrdval: Value=KOUTP_CCCtrlSta_enum_ovrdval
  VVMC_CCMSASpdWar_flg_Inproc : FVT_lib/outp/OverrideAndLimit  SystemSampleTime=-1  VariantActivationTime=update diagram  Latency=0  AutoFrameSizeCalculation=off
      link override Signal_Limit/_maxval: Value=KOUTP_CCMSASpdWar_flg_maxval
      link override Signal_Limit/_minval: Value=KOUTP_CCMSASpdWar_flg_minval
      link override Signal_Override/_ovrdflg: Value=KOUTP_CCMSASpdWar_flg_ovrdflg
      link override Signal_Override/_ovrdval: Value=KOUTP_CCMSASpdWar_flg_ovrdval
  VVMC_CalibratedAccX_G_Inproc : FVT_lib/outp/OverrideAndLimit  SystemSampleTime=-1  VariantActivationTime=update diagram  Latency=0  AutoFrameSizeCalculation=off
      link override Signal_Limit/_maxval: Value=KOUTP_CalibratedAccX_G_maxval
      link override Signal_Limit/_minval: Value=KOUTP_CalibratedAccX_G_minval
      link override Signal_Override/_ovrdflg: Value=KOUTP_CalibratedAccX_G_ovrdflg
      link override Signal_Override/_ovrdval: Value=KOUTP_CalibratedAccX_G_ovrdval
  VVMC_CalibratedAccY_G_Inproc : FVT_lib/outp/OverrideAndLimit  SystemSampleTime=-1  VariantActivationTime=update diagram  Latency=0  AutoFrameSizeCalculation=off
      link override Signal_Limit/_maxval: Value=KOUTP_CalibratedAccY_G_maxval
      link override Signal_Limit/_minval: Value=KOUTP_CalibratedAccY_G_minval
      link override Signal_Override/_ovrdflg: Value=KOUTP_CalibratedAccY_G_ovrdflg
      link override Signal_Override/_ovrdval: Value=KOUTP_CalibratedAccY_G_ovrdval
  VVMC_CalibratedAccZ_G_Inproc : FVT_lib/outp/OverrideAndLimit  SystemSampleTime=-1  VariantActivationTime=update diagram  Latency=0  AutoFrameSizeCalculation=off
      link override Signal_Limit/_maxval: Value=KOUTP_CalibratedAccZ_G_maxval
      link override Signal_Limit/_minval: Value=KOUTP_CalibratedAccZ_G_minval
      link override Signal_Override/_ovrdflg: Value=KOUTP_CalibratedAccZ_G_ovrdflg
      link override Signal_Override/_ovrdval: Value=KOUTP_CalibratedAccZ_G_ovrdval
  VVMC_CalibratedGyroX_Dps_Inproc : FVT_lib/outp/OverrideAndLimit  SystemSampleTime=-1  VariantActivationTime=update diagram  Latency=0  AutoFrameSizeCalculation=off
      link override Signal_Limit/_maxval: Value=KOUTP_CalibratedGyroX_Dps_maxval
      link override Signal_Limit/_minval: Value=KOUTP_CalibratedGyroX_Dps_minval
      link override Signal_Override/_ovrdflg: Value=KOUTP_CalibratedGyroX_Dps_ovrdflg
      link override Signal_Override/_ovrdval: Value=KOUTP_CalibratedGyroX_Dps_ovrdval
  VVMC_CalibratedGyroY_Dps_Inproc : FVT_lib/outp/OverrideAndLimit  SystemSampleTime=-1  VariantActivationTime=update diagram  Latency=0  AutoFrameSizeCalculation=off
      link override Signal_Limit/_maxval: Value=KOUTP_CalibratedGyroY_Dps_maxval
      link override Signal_Limit/_minval: Value=KOUTP_CalibratedGyroY_Dps_minval
      link override Signal_Override/_ovrdflg: Value=KOUTP_CalibratedGyroY_Dps_ovrdflg
      link override Signal_Override/_ovrdval: Value=KOUTP_CalibratedGyroY_Dps_ovrdval
  VVMC_CalibratedGyroZ_Dps_Inproc : FVT_lib/outp/OverrideAndLimit  SystemSampleTime=-1  VariantActivationTime=update diagram  Latency=0  AutoFrameSizeCalculation=off
      link override Signal_Limit/_maxval: Value=KOUTP_CalibratedGyroZ_Dps_maxval
      link override Signal_Limit/_minval: Value=KOUTP_CalibratedGyroZ_Dps_minval
      link override Signal_Override/_ovrdflg: Value=KOUTP_CalibratedGyroZ_Dps_ovrdflg
      link override Signal_Override/_ovrdval: Value=KOUTP_CalibratedGyroZ_Dps_ovrdval
  VVMC_DISCReqAcc_mps2_Inproc : FVT_lib/outp/OverrideAndLimit  SystemSampleTime=-1  VariantActivationTime=update diagram  Latency=0  AutoFrameSizeCalculation=off
      link override Signal_Limit/_maxval: Value=KOUTP_DISCReqAcc_mps2_maxval
      link override Signal_Limit/_minval: Value=KOUTP_DISCReqAcc_mps2_minval
      link override Signal_Override/_ovrdflg: Value=KOUTP_DISCReqAcc_mps2_ovrdflg
      link override Signal_Override/_ovrdval: Value=KOUTP_DISCReqAcc_mps2_ovrdval
  VVMC_ExtraMSACtrlSta_enum_Inproc : FVT_lib/outp/OverrideAndLimit  SystemSampleTime=-1  VariantActivationTime=update diagram  Latency=0  AutoFrameSizeCalculation=off
      link override Signal_Limit/_maxval: Value=KOUTP_ExtraMSACtrlSta_enum_maxval
      link override Signal_Limit/_minval: Value=KOUTP_ExtraMSACtrlSta_enum_minval
      link override Signal_Override/_ovrdflg: Value=KOUTP_ExtraMSACtrlSta_enum_ovrdflg
      link override Signal_Override/_ovrdval: Value=KOUTP_ExtraMSACtrlSta_enum_ovrdval
  VVMC_FCMACCmode_enum_Inproc : FVT_lib/outp/OverrideAndLimit  SystemSampleTime=-1  VariantActivationTime=update diagram  Latency=0  AutoFrameSizeCalculation=off
      link override Signal_Limit/_maxval: Value=KOUTP_FCMACCmode_enum_maxval
      link override Signal_Limit/_minval: Value=KOUTP_FCMACCmode_enum_minval
      link override Signal_Override/_ovrdflg: Value=KOUTP_FCMACCmode_enum_ovrdflg
      link override Signal_Override/_ovrdval: Value=KOUTP_FCMACCmode_enum_ovrdval
  VVMC_FCMLDWFault_flg_Inproc : FVT_lib/outp/OverrideAndLimit  SystemSampleTime=-1  VariantActivationTime=update diagram  Latency=0  AutoFrameSizeCalculation=off
      link override Signal_Limit/_maxval: Value=KOUTP_FCMLDWFault_flg_maxval
      link override Signal_Limit/_minval: Value=KOUTP_FCMLDWFault_flg_minval
      link override Signal_Override/_ovrdflg: Value=KOUTP_FCMLDWFault_flg_ovrdflg
      link override Signal_Override/_ovrdval: Value=KOUTP_FCMLDWFault_flg_ovrdval
  VVMC_FCMLDWRequest_enum_Inproc : FVT_lib/outp/OverrideAndLimit  SystemSampleTime=-1  VariantActivationTime=update diagram  Latency=0  AutoFrameSizeCalculation=off
      link override Signal_Limit/_maxval: Value=KOUTP_FCMLDWRequest_enum_maxval
      link override Signal_Limit/_minval: Value=KOUTP_FCMLDWRequest_enum_minval
      link override Signal_Override/_ovrdflg: Value=KOUTP_FCMLDWRequest_enum_ovrdflg
      link override Signal_Override/_ovrdval: Value=KOUTP_FCMLDWRequest_enum_ovrdval
  VVMC_FDCVMCAPSAngleTarget_deg_Inproc : FVT_lib/outp/OverrideAndLimit  SystemSampleTime=-1  VariantActivationTime=update diagram  Latency=0  AutoFrameSizeCalculation=off
      link override Signal_Limit/_maxval: Value=KOUTP_FDCVMCAPSAngleTarget_deg_maxval
      link override Signal_Limit/_minval: Value=KOUTP_FDCVMCAPSAngleTarget_deg_minval
      link override Signal_Override/_ovrdflg: Value=KOUTP_FDCVMCAPSAngleTarget_deg_ovrdflg
      link override Signal_Override/_ovrdval: Value=KOUTP_FDCVMCAPSAngleTarget_deg_ovrdval
  VVMC_FDCVMCAPSRqEPSCtrl_flg_Inproc : FVT_lib/outp/OverrideAndLimit  SystemSampleTime=-1  VariantActivationTime=update diagram  Latency=0  AutoFrameSizeCalculation=off
      link override Signal_Limit/_maxval: Value=KOUTP_FDCVMCAPSRqEPSCtrl_flg_maxval
      link override Signal_Limit/_minval: Value=KOUTP_FDCVMCAPSRqEPSCtrl_flg_minval
      link override Signal_Override/_ovrdflg: Value=KOUTP_FDCVMCAPSRqEPSCtrl_flg_ovrdflg
      link override Signal_Override/_ovrdval: Value=KOUTP_FDCVMCAPSRqEPSCtrl_flg_ovrdval
  VVMC_FDCVMCAPSVRqEPSCtrl_flg_Inproc : FVT_lib/outp/OverrideAndLimit  SystemSampleTime=-1  VariantActivationTime=update diagram  Latency=0  AutoFrameSizeCalculation=off
      link override Signal_Limit/_maxval: Value=KOUTP_FDCVMCAPSVRqEPSCtrl_flg_maxval
      link override Signal_Limit/_minval: Value=KOUTP_FDCVMCAPSVRqEPSCtrl_flg_minval
      link override Signal_Override/_ovrdflg: Value=KOUTP_FDCVMCAPSVRqEPSCtrl_flg_ovrdflg
      link override Signal_Override/_ovrdval: Value=KOUTP_FDCVMCAPSVRqEPSCtrl_flg_ovrdval
  VVMC_FDCVMCAngCtrlTqWtGn_pct_Inproc : FVT_lib/outp/OverrideAndLimit  SystemSampleTime=-1  VariantActivationTime=update diagram  Latency=0  AutoFrameSizeCalculation=off
      link override Signal_Limit/_maxval: Value=KOUTP_FDCVMCAngCtrlTqWtGn_pct_maxval
      link override Signal_Limit/_minval: Value=KOUTP_FDCVMCAngCtrlTqWtGn_pct_minval
      link override Signal_Override/_ovrdflg: Value=KOUTP_FDCVMCAngCtrlTqWtGn_pct_ovrdflg
      link override Signal_Override/_ovrdval: Value=KOUTP_FDCVMCAngCtrlTqWtGn_pct_ovrdval
  VVMC_FDCVMCDrInpTqBstAct_flg_Inproc : FVT_lib/outp/OverrideAndLimit  SystemSampleTime=-1  VariantActivationTime=update diagram  Latency=0  AutoFrameSizeCalculation=off
      link override Signal_Limit/_maxval: Value=KOUTP_FDCVMCDrInpTqBstAct_flg_maxval
      link override Signal_Limit/_minval: Value=KOUTP_FDCVMCDrInpTqBstAct_flg_minval
      link override Signal_Override/_ovrdflg: Value=KOUTP_FDCVMCDrInpTqBstAct_flg_ovrdflg
      link override Signal_Override/_ovrdval: Value=KOUTP_FDCVMCDrInpTqBstAct_flg_ovrdval
  VVMC_FDCVMCDrInpTqBstGn_pct_Inproc : FVT_lib/outp/OverrideAndLimit  SystemSampleTime=-1  VariantActivationTime=update diagram  Latency=0  AutoFrameSizeCalculation=off
      link override Signal_Limit/_maxval: Value=KOUTP_FDCVMCDrInpTqBstGn_pct_maxval
      link override Signal_Limit/_minval: Value=KOUTP_FDCVMCDrInpTqBstGn_pct_minval
      link override Signal_Override/_ovrdflg: Value=KOUTP_FDCVMCDrInpTqBstGn_pct_ovrdflg
      link override Signal_Override/_ovrdval: Value=KOUTP_FDCVMCDrInpTqBstGn_pct_ovrdval
  VVMC_FDCVMCMaxAngCtrlOutTqLim_Nm_Inproc : FVT_lib/outp/OverrideAndLimit  SystemSampleTime=-1  VariantActivationTime=update diagram  Latency=0  AutoFrameSizeCalculation=off
      link override Signal_Limit/_maxval: Value=KOUTP_FDCVMCMaxAngCtrlOutTqLim_Nm_maxval
      link override Signal_Limit/_minval: Value=KOUTP_FDCVMCMaxAngCtrlOutTqLim_Nm_minval
      link override Signal_Override/_ovrdflg: Value=KOUTP_FDCVMCMaxAngCtrlOutTqLim_Nm_ovrdflg
      link override Signal_Override/_ovrdval: Value=KOUTP_FDCVMCMaxAngCtrlOutTqLim_Nm_ovrdval
  VVMC_FeatArbitrFinal_enum_Inproc : FVT_lib/outp/OverrideAndLimit  SystemSampleTime=-1  VariantActivationTime=update diagram  Latency=0  AutoFrameSizeCalculation=off
      link override Signal_Limit/_maxval: Value=KOUTP_FeatArbitrFinal_enum_maxval
      link override Signal_Limit/_minval: Value=KOUTP_FeatArbitrFinal_enum_minval
      link override Signal_Override/_ovrdflg: Value=KOUTP_FeatArbitrFinal_enum_ovrdflg
      link override Signal_Override/_ovrdval: Value=KOUTP_FeatArbitrFinal_enum_ovrdval
  VVMC_FeatArbitrSta_enum_Inproc : FVT_lib/outp/OverrideAndLimit  SystemSampleTime=-1  VariantActivationTime=update diagram  Latency=0  AutoFrameSizeCalculation=off
      link override Signal_Limit/_maxval: Value=KOUTP_FeatArbitrSta_enum_maxval
      link override Signal_Limit/_minval: Value=KOUTP_FeatArbitrSta_enum_minval
      link override Signal_Override/_ovrdflg: Value=KOUTP_FeatArbitrSta_enum_ovrdflg
      link override Signal_Override/_ovrdval: Value=KOUTP_FeatArbitrSta_enum_ovrdval
  VVMC_FeatReqSpd_kph_Inproc : FVT_lib/outp/OverrideAndLimit  SystemSampleTime=-1  VariantActivationTime=update diagram  Latency=0  AutoFrameSizeCalculation=off
      link override Signal_Limit/_maxval: Value=KOUTP_FeatReqSpd_kph_maxval
      link override Signal_Limit/_minval: Value=KOUTP_FeatReqSpd_kph_minval
      link override Signal_Override/_ovrdflg: Value=KOUTP_FeatReqSpd_kph_ovrdflg
      link override Signal_Override/_ovrdval: Value=KOUTP_FeatReqSpd_kph_ovrdval
  VVMC_FeatSetSpdFinal_raw32_Inproc : FVT_lib/outp/OverrideAndLimit  SystemSampleTime=-1  VariantActivationTime=update diagram  Latency=0  AutoFrameSizeCalculation=off
      link override Signal_Limit/_maxval: Value=KOUTP_FeatSetSpdFinal_raw32_maxval
      link override Signal_Limit/_minval: Value=KOUTP_FeatSetSpdFinal_raw32_minval
      link override Signal_Override/_ovrdflg: Value=KOUTP_FeatSetSpdFinal_raw32_ovrdflg
      link override Signal_Override/_ovrdval: Value=KOUTP_FeatSetSpdFinal_raw32_ovrdval
  VVMC_ForceLowBeam_enum_Inproc : FVT_lib/outp/OverrideAndLimit  SystemSampleTime=-1  VariantActivationTime=update diagram  Latency=0  AutoFrameSizeCalculation=off
      link override Signal_Limit/_maxval: Value=KOUTP_ForceLowBeam_enum_maxval
      link override Signal_Limit/_minval: Value=KOUTP_ForceLowBeam_enum_minval
      link override Signal_Override/_ovrdflg: Value=KOUTP_ForceLowBeam_enum_ovrdflg
      link override Signal_Override/_ovrdval: Value=KOUTP_ForceLowBeam_enum_ovrdval
  VVMC_FrontRearSlipRatioCtrl_flg_Inproc : FVT_lib/outp/OverrideAndLimit  SystemSampleTime=-1  VariantActivationTime=update diagram  Latency=0  AutoFrameSizeCalculation=off
      link override Signal_Limit/_maxval: Value=KOUTP_FrontRearSlipRatioCtrl_flg_maxval
      link override Signal_Limit/_minval: Value=KOUTP_FrontRearSlipRatioCtrl_flg_minval
      link override Signal_Override/_ovrdflg: Value=KOUTP_FrontRearSlipRatioCtrl_flg_ovrdflg
      link override Signal_Override/_ovrdval: Value=KOUTP_FrontRearSlipRatioCtrl_flg_ovrdval
  VVMC_HazardWarningReq_flg_Inproc : FVT_lib/outp/OverrideAndLimit  SystemSampleTime=-1  VariantActivationTime=update diagram  Latency=0  AutoFrameSizeCalculation=off
      link override Signal_Limit/_maxval: Value=KOUTP_HazardWarningReq_flg_maxval
      link override Signal_Limit/_minval: Value=KOUTP_HazardWarningReq_flg_minval
      link override Signal_Override/_ovrdflg: Value=KOUTP_HazardWarningReq_flg_ovrdflg
      link override Signal_Override/_ovrdval: Value=KOUTP_HazardWarningReq_flg_ovrdval
  VVMC_IMUEnaCmd_flg_Inproc : FVT_lib/outp/OverrideAndLimit  SystemSampleTime=-1  VariantActivationTime=update diagram  Latency=0  AutoFrameSizeCalculation=off
      link override Signal_Limit/_maxval: Value=KOUTP_IMUEnaCmd_flg_maxval
      link override Signal_Limit/_minval: Value=KOUTP_IMUEnaCmd_flg_minval
      link override Signal_Override/_ovrdflg: Value=KOUTP_IMUEnaCmd_flg_ovrdflg
      link override Signal_Override/_ovrdval: Value=KOUTP_IMUEnaCmd_flg_ovrdval
  VVMC_ISOAccLimit_mps2_Inproc : FVT_lib/outp/OverrideAndLimit  SystemSampleTime=-1  VariantActivationTime=update diagram  Latency=0  AutoFrameSizeCalculation=off
      link override Signal_Limit/_maxval: Value=KOUTP_ISOAccLimit_mps2_maxval
      link override Signal_Limit/_minval: Value=KOUTP_ISOAccLimit_mps2_minval
      link override Signal_Override/_ovrdflg: Value=KOUTP_ISOAccLimit_mps2_ovrdflg
      link override Signal_Override/_ovrdval: Value=KOUTP_ISOAccLimit_mps2_ovrdval
  VVMC_ISODecLimit_mps2_Inproc : FVT_lib/outp/OverrideAndLimit  SystemSampleTime=-1  VariantActivationTime=update diagram  Latency=0  AutoFrameSizeCalculation=off
      link override Signal_Limit/_maxval: Value=KOUTP_ISODecLimit_mps2_maxval
      link override Signal_Limit/_minval: Value=KOUTP_ISODecLimit_mps2_minval
      link override Signal_Override/_ovrdflg: Value=KOUTP_ISODecLimit_mps2_ovrdflg
      link override Signal_Override/_ovrdval: Value=KOUTP_ISODecLimit_mps2_ovrdval
  VVMC_ISOJerkLimit_mps3_Inproc : FVT_lib/outp/OverrideAndLimit  SystemSampleTime=-1  VariantActivationTime=update diagram  Latency=0  AutoFrameSizeCalculation=off
      link override Signal_Limit/_maxval: Value=KOUTP_ISOJerkLimit_mps3_maxval
      link override Signal_Limit/_minval: Value=KOUTP_ISOJerkLimit_mps3_minval
      link override Signal_Override/_ovrdflg: Value=KOUTP_ISOJerkLimit_mps3_ovrdflg
      link override Signal_Override/_ovrdval: Value=KOUTP_ISOJerkLimit_mps3_ovrdval
  VVMC_JerkPCT_pct_Inproc : FVT_lib/outp/OverrideAndLimit  SystemSampleTime=-1  VariantActivationTime=update diagram  Latency=0  AutoFrameSizeCalculation=off
      link override Signal_Limit/_maxval: Value=KOUTP_JerkPCT_pct_maxval
      link override Signal_Limit/_minval: Value=KOUTP_JerkPCT_pct_minval
      link override Signal_Override/_ovrdflg: Value=KOUTP_JerkPCT_pct_ovrdflg
      link override Signal_Override/_ovrdval: Value=KOUTP_JerkPCT_pct_ovrdval
  VVMC_LKAHODDisplayWarning_flg_Inproc : FVT_lib/outp/OverrideAndLimit  SystemSampleTime=-1  VariantActivationTime=update diagram  Latency=0  AutoFrameSizeCalculation=off
      link override Signal_Limit/_maxval: Value=KOUTP_LKAHODDisplayWarning_flg_maxval
      link override Signal_Limit/_minval: Value=KOUTP_LKAHODDisplayWarning_flg_minval
      link override Signal_Override/_ovrdflg: Value=KOUTP_LKAHODDisplayWarning_flg_ovrdflg
      link override Signal_Override/_ovrdval: Value=KOUTP_LKAHODDisplayWarning_flg_ovrdval
  VVMC_LKAHODSoundWarning_flg_Inproc : FVT_lib/outp/OverrideAndLimit  SystemSampleTime=-1  VariantActivationTime=update diagram  Latency=0  AutoFrameSizeCalculation=off
      link override Signal_Limit/_maxval: Value=KOUTP_LKAHODSoundWarning_flg_maxval
      link override Signal_Limit/_minval: Value=KOUTP_LKAHODSoundWarning_flg_minval
      link override Signal_Override/_ovrdflg: Value=KOUTP_LKAHODSoundWarning_flg_ovrdflg
      link override Signal_Override/_ovrdval: Value=KOUTP_LKAHODSoundWarning_flg_ovrdval
  VVMC_LKAStrToqReq_Nm_Inproc : FVT_lib/outp/OverrideAndLimit  SystemSampleTime=-1  VariantActivationTime=update diagram  Latency=0  AutoFrameSizeCalculation=off
      link override Signal_Limit/_maxval: Value=KOUTP_LKAStrToqReq_Nm_maxval
      link override Signal_Limit/_minval: Value=KOUTP_LKAStrToqReq_Nm_minval
      link override Signal_Override/_ovrdflg: Value=KOUTP_LKAStrToqReq_Nm_ovrdflg
      link override Signal_Override/_ovrdval: Value=KOUTP_LKAStrToqReq_Nm_ovrdval
  VVMC_LKATOIAct_enum_Inproc : FVT_lib/outp/OverrideAndLimit  SystemSampleTime=-1  VariantActivationTime=update diagram  Latency=0  AutoFrameSizeCalculation=off
      link override Signal_Limit/_maxval: Value=KOUTP_LKATOIAct_enum_maxval
      link override Signal_Limit/_minval: Value=KOUTP_LKATOIAct_enum_minval
      link override Signal_Override/_ovrdflg: Value=KOUTP_LKATOIAct_enum_ovrdflg
      link override Signal_Override/_ovrdval: Value=KOUTP_LKATOIAct_enum_ovrdval
  VVMC_LKATOIFault_flg_Inproc : FVT_lib/outp/OverrideAndLimit  SystemSampleTime=-1  VariantActivationTime=update diagram  Latency=0  AutoFrameSizeCalculation=off
      link override Signal_Limit/_maxval: Value=KOUTP_LKATOIFault_flg_maxval
      link override Signal_Limit/_minval: Value=KOUTP_LKATOIFault_flg_minval
      link override Signal_Override/_ovrdflg: Value=KOUTP_LKATOIFault_flg_ovrdflg
      link override Signal_Override/_ovrdval: Value=KOUTP_LKATOIFault_flg_ovrdval
  VVMC_LVDAACCStatusInformation_flg_Inproc : FVT_lib/outp/OverrideAndLimit  SystemSampleTime=-1  VariantActivationTime=update diagram  Latency=0  AutoFrameSizeCalculation=off
      link override Signal_Limit/_maxval: Value=KOUTP_LVDAACCStatusInformation_flg_maxval
      link override Signal_Limit/_minval: Value=KOUTP_LVDAACCStatusInformation_flg_minval
      link override Signal_Override/_ovrdflg: Value=KOUTP_LVDAACCStatusInformation_flg_ovrdflg
      link override Signal_Override/_ovrdval: Value=KOUTP_LVDAACCStatusInformation_flg_ovrdval
  VVMC_LVDADisabled_flg_Inproc : FVT_lib/outp/OverrideAndLimit  SystemSampleTime=-1  VariantActivationTime=update diagram  Latency=0  AutoFrameSizeCalculation=off
      link override Signal_Limit/_maxval: Value=KOUTP_LVDADisabled_flg_maxval
      link override Signal_Limit/_minval: Value=KOUTP_LVDADisabled_flg_minval
      link override Signal_Override/_ovrdflg: Value=KOUTP_LVDADisabled_flg_ovrdflg
      link override Signal_Override/_ovrdval: Value=KOUTP_LVDADisabled_flg_ovrdval
  VVMC_LVDAFailinfo_flg_Inproc : FVT_lib/outp/OverrideAndLimit  SystemSampleTime=-1  VariantActivationTime=update diagram  Latency=0  AutoFrameSizeCalculation=off
      link override Signal_Limit/_maxval: Value=KOUTP_LVDAFailinfo_flg_maxval
      link override Signal_Limit/_minval: Value=KOUTP_LVDAFailinfo_flg_minval
      link override Signal_Override/_ovrdflg: Value=KOUTP_LVDAFailinfo_flg_ovrdflg
      link override Signal_Override/_ovrdval: Value=KOUTP_LVDAFailinfo_flg_ovrdval
  VVMC_LVDAMuteSta_enum_Inproc : FVT_lib/outp/OverrideAndLimit  SystemSampleTime=-1  VariantActivationTime=update diagram  Latency=0  AutoFrameSizeCalculation=off
      link override Signal_Limit/_maxval: Value=KOUTP_LVDAMuteSta_enum_maxval
      link override Signal_Limit/_minval: Value=KOUTP_LVDAMuteSta_enum_minval
      link override Signal_Override/_ovrdflg: Value=KOUTP_LVDAMuteSta_enum_ovrdflg
      link override Signal_Override/_ovrdval: Value=KOUTP_LVDAMuteSta_enum_ovrdval
  VVMC_LVDAWarning_flg_Inproc : FVT_lib/outp/OverrideAndLimit  SystemSampleTime=-1  VariantActivationTime=update diagram  Latency=0  AutoFrameSizeCalculation=off
      link override Signal_Limit/_maxval: Value=KOUTP_LVDAWarning_flg_maxval
      link override Signal_Limit/_minval: Value=KOUTP_LVDAWarning_flg_minval
      link override Signal_Override/_ovrdflg: Value=KOUTP_LVDAWarning_flg_ovrdflg
      link override Signal_Override/_ovrdval: Value=KOUTP_LVDAWarning_flg_ovrdval
  VVMC_LatAccCtrl_flg_Inproc : FVT_lib/outp/OverrideAndLimit  SystemSampleTime=-1  VariantActivationTime=update diagram  Latency=0  AutoFrameSizeCalculation=off
      link override Signal_Limit/_maxval: Value=KOUTP_LatAccCtrl_flg_maxval
      link override Signal_Limit/_minval: Value=KOUTP_LatAccCtrl_flg_minval
      link override Signal_Override/_ovrdflg: Value=KOUTP_LatAccCtrl_flg_ovrdflg
      link override Signal_Override/_ovrdval: Value=KOUTP_LatAccCtrl_flg_ovrdval
  VVMC_LateralCtrl_flg_Inproc : FVT_lib/outp/OverrideAndLimit  SystemSampleTime=-1  VariantActivationTime=update diagram  Latency=0  AutoFrameSizeCalculation=off
      link override Signal_Limit/_maxval: Value=KOUTP_LateralCtrl_flg_maxval
      link override Signal_Limit/_minval: Value=KOUTP_LateralCtrl_flg_minval
      link override Signal_Override/_ovrdflg: Value=KOUTP_LateralCtrl_flg_ovrdflg
      link override Signal_Override/_ovrdval: Value=KOUTP_LateralCtrl_flg_ovrdval
  VVMC_LeftTurnLightReq_flg_Inproc : FVT_lib/outp/OverrideAndLimit  SystemSampleTime=-1  VariantActivationTime=update diagram  Latency=0  AutoFrameSizeCalculation=off
      link override Signal_Limit/_maxval: Value=KOUTP_LeftTurnLightReq_flg_maxval
      link override Signal_Limit/_minval: Value=KOUTP_LeftTurnLightReq_flg_minval
      link override Signal_Override/_ovrdflg: Value=KOUTP_LeftTurnLightReq_flg_ovrdflg
      link override Signal_Override/_ovrdval: Value=KOUTP_LeftTurnLightReq_flg_ovrdval
  VVMC_LimitPCT_pct_Inproc : FVT_lib/outp/OverrideAndLimit  SystemSampleTime=-1  VariantActivationTime=update diagram  Latency=0  AutoFrameSizeCalculation=off
      link override Signal_Limit/_maxval: Value=KOUTP_LimitPCT_pct_maxval
      link override Signal_Limit/_minval: Value=KOUTP_LimitPCT_pct_minval
      link override Signal_Override/_ovrdflg: Value=KOUTP_LimitPCT_pct_ovrdflg
      link override Signal_Override/_ovrdval: Value=KOUTP_LimitPCT_pct_ovrdval
  VVMC_LongAcc_Gps_Inproc : FVT_lib/outp/OverrideAndLimit  SystemSampleTime=-1  VariantActivationTime=update diagram  Latency=0  AutoFrameSizeCalculation=off
      link override Signal_Limit/_maxval: Value=KOUTP_LongAcc_Gps_maxval
      link override Signal_Limit/_minval: Value=KOUTP_LongAcc_Gps_minval
      link override Signal_Override/_ovrdflg: Value=KOUTP_LongAcc_Gps_ovrdflg
      link override Signal_Override/_ovrdval: Value=KOUTP_LongAcc_Gps_ovrdval
  VVMC_MSACtrlSta_enum_Inproc : FVT_lib/outp/OverrideAndLimit  SystemSampleTime=-1  VariantActivationTime=update diagram  Latency=0  AutoFrameSizeCalculation=off
      link override Signal_Limit/_maxval: Value=KOUTP_MSACtrlSta_enum_maxval
      link override Signal_Limit/_minval: Value=KOUTP_MSACtrlSta_enum_minval
      link override Signal_Override/_ovrdflg: Value=KOUTP_MSACtrlSta_enum_ovrdflg
      link override Signal_Override/_ovrdval: Value=KOUTP_MSACtrlSta_enum_ovrdval
  VVMC_MeterIndSpeed_raw32_Inproc : FVT_lib/outp/OverrideAndLimit  SystemSampleTime=-1  VariantActivationTime=update diagram  Latency=0  AutoFrameSizeCalculation=off
      link override Signal_Limit/_maxval: Value=KOUTP_MeterIndSpeed_raw32_maxval
      link override Signal_Limit/_minval: Value=KOUTP_MeterIndSpeed_raw32_minval
      link override Signal_Override/_ovrdflg: Value=KOUTP_MeterIndSpeed_raw32_ovrdflg
      link override Signal_Override/_ovrdval: Value=KOUTP_MeterIndSpeed_raw32_ovrdval
  VVMC_RearWhlSlipRatioCtrl_flg_Inproc : FVT_lib/outp/OverrideAndLimit  SystemSampleTime=-1  VariantActivationTime=update diagram  Latency=0  AutoFrameSizeCalculation=off
      link override Signal_Limit/_maxval: Value=KOUTP_RearWhlSlipRatioCtrl_flg_maxval
      link override Signal_Limit/_minval: Value=KOUTP_RearWhlSlipRatioCtrl_flg_minval
      link override Signal_Override/_ovrdflg: Value=KOUTP_RearWhlSlipRatioCtrl_flg_ovrdflg
      link override Signal_Override/_ovrdval: Value=KOUTP_RearWhlSlipRatioCtrl_flg_ovrdval
  VVMC_RightTurnLightReq_flg_Inproc : FVT_lib/outp/OverrideAndLimit  SystemSampleTime=-1  VariantActivationTime=update diagram  Latency=0  AutoFrameSizeCalculation=off
      link override Signal_Limit/_maxval: Value=KOUTP_RightTurnLightReq_flg_maxval
      link override Signal_Limit/_minval: Value=KOUTP_RightTurnLightReq_flg_minval
      link override Signal_Override/_ovrdflg: Value=KOUTP_RightTurnLightReq_flg_ovrdflg
      link override Signal_Override/_ovrdval: Value=KOUTP_RightTurnLightReq_flg_ovrdval
  VVMC_SPD2ACCAct_flg_Inproc : FVT_lib/outp/OverrideAndLimit  SystemSampleTime=-1  VariantActivationTime=update diagram  Latency=0  AutoFrameSizeCalculation=off
      link override Signal_Limit/_maxval: Value=KOUTP_SPD2ACCAct_flg_maxval
      link override Signal_Limit/_minval: Value=KOUTP_SPD2ACCAct_flg_minval
      link override Signal_Override/_ovrdflg: Value=KOUTP_SPD2ACCAct_flg_ovrdflg
      link override Signal_Override/_ovrdval: Value=KOUTP_SPD2ACCAct_flg_ovrdval
  VVMC_SafetyCtrl_flg_Inproc : FVT_lib/outp/OverrideAndLimit  SystemSampleTime=-1  VariantActivationTime=update diagram  Latency=0  AutoFrameSizeCalculation=off
      link override Signal_Limit/_maxval: Value=KOUTP_SafetyCtrl_flg_maxval
      link override Signal_Limit/_minval: Value=KOUTP_SafetyCtrl_flg_minval
      link override Signal_Override/_ovrdflg: Value=KOUTP_SafetyCtrl_flg_ovrdflg
      link override Signal_Override/_ovrdval: Value=KOUTP_SafetyCtrl_flg_ovrdval
  VVMC_SingleWhlSlipRatioCtrl_flg_Inproc : FVT_lib/outp/OverrideAndLimit  SystemSampleTime=-1  VariantActivationTime=update diagram  Latency=0  AutoFrameSizeCalculation=off
      link override Signal_Limit/_maxval: Value=KOUTP_SingleWhlSlipRatioCtrl_flg_maxval
      link override Signal_Limit/_minval: Value=KOUTP_SingleWhlSlipRatioCtrl_flg_minval
      link override Signal_Override/_ovrdflg: Value=KOUTP_SingleWhlSlipRatioCtrl_flg_ovrdflg
      link override Signal_Override/_ovrdval: Value=KOUTP_SingleWhlSlipRatioCtrl_flg_ovrdval
  VVMC_TargetType_enum_Inproc : FVT_lib/outp/OverrideAndLimit  SystemSampleTime=-1  VariantActivationTime=update diagram  Latency=0  AutoFrameSizeCalculation=off
      link override Signal_Limit/_maxval: Value=KOUTP_TargetType_enum_maxval
      link override Signal_Limit/_minval: Value=KOUTP_TargetType_enum_minval
      link override Signal_Override/_ovrdflg: Value=KOUTP_TargetType_enum_ovrdflg
      link override Signal_Override/_ovrdval: Value=KOUTP_TargetType_enum_ovrdval
  VVMC_TimeGapCalcu_s_Inproc : FVT_lib/outp/OverrideAndLimit  SystemSampleTime=-1  VariantActivationTime=update diagram  Latency=0  AutoFrameSizeCalculation=off
      link override Signal_Limit/_maxval: Value=KOUTP_TimeGapCalcu_s_maxval
      link override Signal_Limit/_minval: Value=KOUTP_TimeGapCalcu_s_minval
      link override Signal_Override/_ovrdflg: Value=KOUTP_TimeGapCalcu_s_ovrdflg
      link override Signal_Override/_ovrdval: Value=KOUTP_TimeGapCalcu_s_ovrdval
  VVMC_TimeGapLevel_enum_Inproc : FVT_lib/outp/OverrideAndLimit  SystemSampleTime=-1  VariantActivationTime=update diagram  Latency=0  AutoFrameSizeCalculation=off
      link override Signal_Limit/_maxval: Value=KOUTP_TimeGapLevel_enum_maxval
      link override Signal_Limit/_minval: Value=KOUTP_TimeGapLevel_enum_minval
      link override Signal_Override/_ovrdflg: Value=KOUTP_TimeGapLevel_enum_ovrdflg
      link override Signal_Override/_ovrdval: Value=KOUTP_TimeGapLevel_enum_ovrdval
  VVMC_VMCACCCtrlAvail_flg_Inproc : FVT_lib/outp/OverrideAndLimit  SystemSampleTime=-1  VariantActivationTime=update diagram  Latency=0  AutoFrameSizeCalculation=off
      link override Signal_Limit/_maxval: Value=KOUTP_VMCACCCtrlAvail_flg_maxval
      link override Signal_Limit/_minval: Value=KOUTP_VMCACCCtrlAvail_flg_minval
      link override Signal_Override/_ovrdflg: Value=KOUTP_VMCACCCtrlAvail_flg_ovrdflg
      link override Signal_Override/_ovrdval: Value=KOUTP_VMCACCCtrlAvail_flg_ovrdval
  VVMC_VMCAEBCtrlAvail_flg_Inproc : FVT_lib/outp/OverrideAndLimit  SystemSampleTime=-1  VariantActivationTime=update diagram  Latency=0  AutoFrameSizeCalculation=off
      link override Signal_Limit/_maxval: Value=KOUTP_VMCAEBCtrlAvail_flg_maxval
      link override Signal_Limit/_minval: Value=KOUTP_VMCAEBCtrlAvail_flg_minval
      link override Signal_Override/_ovrdflg: Value=KOUTP_VMCAEBCtrlAvail_flg_ovrdflg
      link override Signal_Override/_ovrdval: Value=KOUTP_VMCAEBCtrlAvail_flg_ovrdval
  VVMC_VMCCCCtrlAvail_flg_Inproc : FVT_lib/outp/OverrideAndLimit  SystemSampleTime=-1  VariantActivationTime=update diagram  Latency=0  AutoFrameSizeCalculation=off
      link override Signal_Limit/_maxval: Value=KOUTP_VMCCCCtrlAvail_flg_maxval
      link override Signal_Limit/_minval: Value=KOUTP_VMCCCCtrlAvail_flg_minval
      link override Signal_Override/_ovrdflg: Value=KOUTP_VMCCCCtrlAvail_flg_ovrdflg
      link override Signal_Override/_ovrdval: Value=KOUTP_VMCCCCtrlAvail_flg_ovrdval
  VVMC_VMCMSACtrlAvail_flg_Inproc : FVT_lib/outp/OverrideAndLimit  SystemSampleTime=-1  VariantActivationTime=update diagram  Latency=0  AutoFrameSizeCalculation=off
      link override Signal_Limit/_maxval: Value=KOUTP_VMCMSACtrlAvail_flg_maxval
      link override Signal_Limit/_minval: Value=KOUTP_VMCMSACtrlAvail_flg_minval
      link override Signal_Override/_ovrdflg: Value=KOUTP_VMCMSACtrlAvail_flg_ovrdflg
      link override Signal_Override/_ovrdval: Value=KOUTP_VMCMSACtrlAvail_flg_ovrdval
  VVMC_VehicleSpeed_kph_Inproc : FVT_lib/outp/OverrideAndLimit  SystemSampleTime=-1  VariantActivationTime=update diagram  Latency=0  AutoFrameSizeCalculation=off
      link override Signal_Limit/_maxval: Value=KOUTP_VehicleSpeed_kph_maxval
      link override Signal_Limit/_minval: Value=KOUTP_VehicleSpeed_kph_minval
      link override Signal_Override/_ovrdflg: Value=KOUTP_VehicleSpeed_kph_ovrdflg
      link override Signal_Override/_ovrdval: Value=KOUTP_VehicleSpeed_kph_ovrdval
  VVMC_VehicleSpeed_mph_Inproc : FVT_lib/outp/OverrideAndLimit  SystemSampleTime=-1  VariantActivationTime=update diagram  Latency=0  AutoFrameSizeCalculation=off
      link override Signal_Limit/_maxval: Value=KOUTP_VehicleSpeed_mph_maxval
      link override Signal_Limit/_minval: Value=KOUTP_VehicleSpeed_mph_minval
      link override Signal_Override/_ovrdflg: Value=KOUTP_VehicleSpeed_mph_ovrdflg
      link override Signal_Override/_ovrdval: Value=KOUTP_VehicleSpeed_mph_ovrdval
  VOUTP_HVTHCMSysAvail_enum : Outport
  VOUTP_LVBattVoltSta_enum : Outport  Port=2
  VOUTP_VehHVPwrAvail4THCM_W : Outport  Port=3
  VOUTP_VehSpeed_kph : Outport  Port=4
  VOUTP_VehSpeedTimeOut_flg : Outport  Port=5
  VOUTP_FSOffSw_enum : Outport  Port=6
  VOUTP_FSOffSwTimeOut_flg : Outport  Port=7
  VOUTP_ChrgPlugSta_enum : Outport  Port=8
  VOUTP_PASDRMR_cm : Outport  Port=9
  VOUTP_PASDRML_cm : Outport  Port=10
  VOUTP_PASDRCR_cm : Outport  Port=11
  VOUTP_PASDRCL_cm : Outport  Port=12
  VOUTP_PASDFMR_cm : Outport  Port=13
  VOUTP_PASDFML_cm : Outport  Port=14
  VOUTP_PASDFCR_cm : Outport  Port=15
  VOUTP_PASDFCL_cm : Outport  Port=16
  VOUTP_APSDRLR_cm : Outport  Port=17
  VOUTP_APSDRLL_cm : Outport  Port=18
  VOUTP_APSDFLR_cm : Outport  Port=19
  VOUTP_APSDFLL_cm : Outport  Port=20
  VOUTP_PASAFCL_enum : Outport  Port=21
  VOUTP_PASARMR_enum : Outport  Port=22
  VOUTP_PASARML_enum : Outport  Port=23
  VOUTP_PASARCR_enum : Outport  Port=24
  VOUTP_PASARCL_enum : Outport  Port=25
  VOUTP_PASAFMR_enum : Outport  Port=26
  VOUTP_PASAFML_enum : Outport  Port=27
  VOUTP_PASAFCR_enum : Outport  Port=28
  VOUTP_USSStaRMR_flg : Outport  Port=29
  VOUTP_USSStaRML_flg : Outport  Port=30
  VOUTP_USSStaRLR_flg : Outport  Port=31
  VOUTP_USSStaRLL_flg : Outport  Port=32
  VOUTP_USSStaRCR_flg : Outport  Port=33
  VOUTP_USSStaRCL_flg : Outport  Port=34
  VOUTP_USSStaFMR_flg : Outport  Port=35
  VOUTP_USSStaFML_flg : Outport  Port=36
  VOUTP_USSStaFLR_flg : Outport  Port=37
  VOUTP_USSStaFLL_flg : Outport  Port=38
  VOUTP_USSStaFCR_flg : Outport  Port=39
  VOUTP_USSStaFCL_flg : Outport  Port=40
  VOUTP_Chime_enum : Outport  Port=41
  VOUTP_SNSRLayout_enum : Outport  Port=42
  VOUTP_StaFSya_flg : Outport  Port=43
  VOUTP_ModOperation_enum : Outport  Port=44
  VOUTP_BrkPedalPos_pct : Outport  Port=45
  VOUTP_BrkPedalPosTimeOut_flg : Outport  Port=46
  VOUTP_LFRawWhlSpeed_kph : Outport  Port=47
  VOUTP_LFRawWhlSpeedTimeOut_flg : Outport  Port=48
  VOUTP_RFRawWhlSpeed_kph : Outport  Port=49
  VOUTP_RFRawWhlSpeedTimeOut_flg : Outport  Port=50
  VOUTP_LRRawWhlSpeed_kph : Outport  Port=51
  VOUTP_LRRawWhlSpeedTimeOut_flg : Outport  Port=52
  VOUTP_RRRawWhlSpeed_kph : Outport  Port=53
  VOUTP_RRRawWhlSpeedTimeOut_flg : Outport  Port=54
  VOUTP_LFRawWhlSpeedV_flg : Outport  Port=55
  VOUTP_LFRawWhlSpeedVTimeOut_flg : Outport  Port=56
  VOUTP_RFRawWhlSpeedV_flg : Outport  Port=57
  VOUTP_RFRawWhlSpeedVTimeOut_flg : Outport  Port=58
  VOUTP_LRRawWhlSpeedV_flg : Outport  Port=59
  VOUTP_LRRawWhlSpeedVTimeOut_flg : Outport  Port=60
  VOUTP_RRRawWhlSpeedV_flg : Outport  Port=61
  VOUTP_RRRawWhlSpeedVTimeOut_flg : Outport  Port=62
  VOUTP_LFWhlRotDir_enum : Outport  Port=63
  VOUTP_LFWhlRotDirTimeOut_flg : Outport  Port=64
  VOUTP_RFWhlRotDir_enum : Outport  Port=65
  VOUTP_RFWhlRotDirTimeOut_flg : Outport  Port=66
  VOUTP_LRWhlRotDir_enum : Outport  Port=67
  VOUTP_LRWhlRotDirTimeOut_flg : Outport  Port=68
  VOUTP_RRWhlRotDir_enum : Outport  Port=69
  VOUTP_RRWhlRotDirTimeOut_flg : Outport  Port=70
  VOUTP_LFPulseCountV_flg : Outport  Port=71
  VOUTP_LFPulseCountVTimeOut_flg : Outport  Port=72
  VOUTP_RFPulseCountV_flg : Outport  Port=73
  VOUTP_RFPulseCountVTimeOut_flg : Outport  Port=74
  VOUTP_LRPulseCountV_flg : Outport  Port=75
  VOUTP_LRPulseCountVTimeOut_flg : Outport  Port=76
  VOUTP_RRPulseCountV_flg : Outport  Port=77
  VOUTP_RRPulseCountVTimeOut_flg : Outport  Port=78
  VOUTP_LFPulseCount_enum : Outport  Port=79
  VOUTP_LFPulseCountTimeOut_flg : Outport  Port=80
  VOUTP_RFPulseCount_enum : Outport  Port=81
  VOUTP_RFPulseCountTimeOut_flg : Outport  Port=82
  VOUTP_LRPulseCount_enum : Outport  Port=83
  VOUTP_LRPulseCountTimeOut_flg : Outport  Port=84
  VOUTP_RRPulseCount_enum : Outport  Port=85
  VOUTP_RRPulseCountTimeOut_flg : Outport  Port=86
  VOUTP_ShifterHandleCmd_enum : Outport  Port=87
  VOUTP_ShifterHandleCmdTimeOut_flg : Outport  Port=88
  VOUTP_DriIntend_enum : Outport  Port=89
  VOUTP_DriIntendTimeOut_flg : Outport  Port=90
  VOUTP_EPSAOIControl_enum : Outport  Port=91
  VOUTP_EPSAOIControlTimeOut_flg : Outport  Port=92
  VOUTP_SASAngle_Deg : Outport  Port=93
  VOUTP_SASAngleTimeOut_flg : Outport  Port=94
  VOUTP_SASSpeed_degps : Outport  Port=95
  VOUTP_SASSpeedTimeOut_flg : Outport  Port=96
  VOUTP_SASSpeedValid_flg : Outport  Port=97
  VOUTP_SASSpeedValidTimeOut_flg : Outport  Port=98
  VOUTP_SASCAL_flg : Outport  Port=99
  VOUTP_SASCALTimeOut_flg : Outport  Port=100
  VOUTP_SASV_flg : Outport  Port=101
  VOUTP_SASVTimeOut_flg : Outport  Port=102
  VOUTP_GRADE_Deg : Outport  Port=103
  VOUTP_GRADETimeOut_flg : Outport  Port=104
  VOUTP_YawRate_degps : Outport  Port=105
  VOUTP_YawRateTimeOut_flg : Outport  Port=106
  VOUTP_LatAccel_Gps : Outport  Port=107
  VOUTP_LatAccelTimeOut_flg : Outport  Port=108
  VOUTP_LongAccel_Gps : Outport  Port=109
  VOUTP_LongAccelTimeOut_flg : Outport  Port=110
  VOUTP_MCPressure_bar : Outport  Port=111
  VOUTP_MCPressureTimeOut_flg : Outport  Port=112
  VOUTP_YawRateV_flg : Outport  Port=113
  VOUTP_YawRateVTimeOut_flg : Outport  Port=114
  VOUTP_LatAccelV_flg : Outport  Port=115
  VOUTP_LatAccelVTimeOut_flg : Outport  Port=116
  VOUTP_LongAccelV_flg : Outport  Port=117
  VOUTP_LongAccelVTimeOut_flg : Outport  Port=118
  VOUTP_MCPressureV_bar : Outport  Port=119
  VOUTP_MCPressureVTimeOut_flg : Outport  Port=120
  VOUTP_BrkSwSta_flg : Outport  Port=121
  VOUTP_BrkSwStaTimeOut_flg : Outport  Port=122
  VOUTP_BrkSwV_flg : Outport  Port=123
  VOUTP_BrkSwVTimeOut_flg : Outport  Port=124
  VOUTP_ESCStandstill_flg : Outport  Port=125
  VOUTP_ESCStandstillTimeOut_flg : Outport  Port=126
  VOUTP_ESCAPSSta_enum : Outport  Port=127
  VOUTP_ESCAPSStaTimeOut_flg : Outport  Port=128
  VOUTP_EPBExtReleaseAvail_flg : Outport  Port=129
  VOUTP_EPBExtReleaseAvailTimeOut_flg : Outport  Port=130
  VOUTP_EPBExtApplyAvail_flg : Outport  Port=131
  VOUTP_EPBExtApplyAvailTimeOut_flg : Outport  Port=132
  VOUTP_EPBErrSta_enum : Outport  Port=133
  VOUTP_EPBErrStaTimeOut_flg : Outport  Port=134
  VOUTP_EPBSta_enum : Outport  Port=135
  VOUTP_EPBStaTimeOut_flg : Outport  Port=136
  VOUTP_AVMparkingcancel_enum : Outport  Port=137
  VOUTP_AVMparkingcancelTimeOut_flg : Outport  Port=138
  VOUTP_AVMparkingexcute_enum : Outport  Port=139
  VOUTP_AVMparkingexcuteTimeOut_flg : Outport  Port=140
  VOUTP_AVMParkingmode_enum : Outport  Port=141
  VOUTP_AVMParkingmodeTimeOut_flg : Outport  Port=142
  VOUTP_AVMErrSTA_flg : Outport  Port=143
  VOUTP_AVMErrSTATimeOut_flg : Outport  Port=144
  VOUTP_IVIStatus_flg : Outport  Port=145
  VOUTP_IVIStatusTimeOut_flg : Outport  Port=146
  VOUTP_CAASSw_enum : Outport  Port=147
  VOUTP_CAASSwTimeOut_flg : Outport  Port=148
  VOUTP_IVIScreen_enum : Outport  Port=149
  VOUTP_IVIScreenTimeOut_flg : Outport  Port=150
  VOUTP_ABSActive_flg : Outport  Port=151
  VOUTP_ABSActiveTimeOut_flg : Outport  Port=152
  VOUTP_TCSActive_flg : Outport  Port=153
  VOUTP_TCSActiveTimeOut_flg : Outport  Port=154
  VOUTP_DriverSeatBeltCmd_flg : Outport  Port=155
  VOUTP_DriverSeatBeltCmdTimeOut_flg : Outport  Port=156
  VOUTP_APSProgressPCT_pct : Outport  Port=157
  VOUTP_APSRQDisplay_enum : Outport  Port=158
  VOUTP_APSSWVer_enum : Outport  Port=159
  VOUTP_APSHWVer_enum : Outport  Port=160
  VOUTP_APSExitCondition_enum : Outport  Port=161
  VOUTP_APSAngleTarget_Deg : Outport  Port=162
  VOUTP_APSVRqEPASCtrl_flg : Outport  Port=163
  VOUTP_APSRqEPASCtrl_flg : Outport  Port=164
  VOUTP_CAASSta_enum : Outport  Port=165
  VOUTP_DKCPDkeyAreaRAPSSta_enum : Outport  Port=166
  VOUTP_DKCParkingModeCmd_enum : Outport  Port=167
  VOUTP_PUIDLowPower_flg : Outport  Port=168
  VOUTP_CAASVMCReqA_flg : Outport  Port=169
  VOUTP_APSShiftPosnReq_enum : Outport  Port=170
  VOUTP_APSSpeedCMD_kph : Outport  Port=171
  VOUTP_APSVMCReqA_flg : Outport  Port=172
  VOUTP_RAPSBCMLamp_enum : Outport  Port=173
  VOUTP_RAPSBCMLockReq_flg : Outport  Port=174
  VOUTP_APSPwrReq_enum : Outport  Port=175
  VOUTP_RAPSErrWarnSta_enum : Outport  Port=176
  VOUTP_RAPSErrLv1_flg : Outport  Port=177
  VOUTP_IVIUserTakeOverAPSSta_flg : Outport  Port=178
  VOUTP_AntitheftSta_enum : Outport  Port=179
  VOUTP_TailgateRemote_enum : Outport  Port=180
  VOUTP_HornCtrl_flg : Outport  Port=181
  VOUTP_AllDoorSW_flg : Outport  Port=182
  VOUTP_BCMDoorLockSta_flg : Outport  Port=183
  VOUTP_AntitheftSeatFlod_flg : Outport  Port=184
  VOUTP_HoodSW_flg : Outport  Port=185
  VOUTP_TailgateSW_flg : Outport  Port=186
  VOUTP_DrDoorSW_flg : Outport  Port=187
  VOUTP_PsDoorSW_flg : Outport  Port=188
  VOUTP_RLDoorSW_flg : Outport  Port=189
  VOUTP_RRDoorSW_flg : Outport  Port=190
  VOUTP_LockSetting_flg : Outport  Port=191
  VOUTP_FrChargingDoorCtrl_enum : Outport  Port=192
  VOUTP_RrChargingDoorCtrl_enum : Outport  Port=193
  VOUTP_CrashDetd_flg : Outport  Port=194
  VOUTP_CTDCtrl_enum : Outport  Port=195
  VOUTP_DoorLockIND_flg : Outport  Port=196
  VOUTP_CTDLockSW_flg : Outport  Port=197
  VOUTP_Dimmer_pct : Outport  Port=198
  VOUTP_DimmerEN_flg : Outport  Port=199
  VOUTP_PosLamp_flg : Outport  Port=200
  VOUTP_LBeam_flg : Outport  Port=201
  VOUTP_HBeam_flg : Outport  Port=202
  VOUTP_RrFogLamp_flg : Outport  Port=203
  VOUTP_BrakeLamp_flg : Outport  Port=204
  VOUTP_ReverseLamp_flg : Outport  Port=205
  VOUTP_LDRL_flg : Outport  Port=206
  VOUTP_RDRL_flg : Outport  Port=207
  VOUTP_LBSD_flg : Outport  Port=208
  VOUTP_RBSD_flg : Outport  Port=209
  VOUTP_HazardSW_flg : Outport  Port=210
  VOUTP_LTurnLP_flg : Outport  Port=211
  VOUTP_RTurnLP_flg : Outport  Port=212
  VOUTP_BCMBuzzerReq_flg : Outport  Port=213
  VOUTP_MirrorCtrl_enum : Outport  Port=214
  VOUTP_MirrorDefog_flg : Outport  Port=215
  VOUTP_RrDefog_flg : Outport  Port=216
  VOUTP_RoomLampH_flg : Outport  Port=217
  VOUTP_RoomLampL_flg : Outport  Port=218
  VOUTP_TrunkRel_flg : Outport  Port=219
  VOUTP_TailgateHDSW_flg : Outport  Port=220
  VOUTP_FrWiperL_flg : Outport  Port=221
  VOUTP_FrWiperH_flg : Outport  Port=222
  VOUTP_RrWiper_flg : Outport  Port=223
  VOUTP_WasherCtrl_enum : Outport  Port=224
  VOUTP_WiperFixMode_flg : Outport  Port=225
  VOUTP_AmbLightBreath1_enum : Outport  Port=226
  VOUTP_AmbLightBreath2_enum : Outport  Port=227
  VOUTP_AmbLightBreath3_enum : Outport  Port=228
  VOUTP_AmbLightBreath4_enum : Outport  Port=229
  VOUTP_AmbLightBreath5_enum : Outport  Port=230
  VOUTP_AmbLightBreath6_enum : Outport  Port=231
  VOUTP_AmbLightBrightness1_enum : Outport  Port=232
  VOUTP_AmbLightBrightness2_enum : Outport  Port=233
  VOUTP_AmbLightBrightness3_enum : Outport  Port=234
  VOUTP_AmbLightBrightness4_enum : Outport  Port=235
  VOUTP_AmbLightBrightness5_enum : Outport  Port=236
  VOUTP_AmbLightBrightness6_enum : Outport  Port=237
  VOUTP_AmbLightColor1_enum : Outport  Port=238
  VOUTP_AmbLightColor2_enum : Outport  Port=239
  VOUTP_AmbLightColor3_enum : Outport  Port=240
  VOUTP_AmbLightColor4_enum : Outport  Port=241
  VOUTP_AmbLightColor5_enum : Outport  Port=242
  VOUTP_AmbLightColor6_enum : Outport  Port=243
  VOUTP_LampPwr_flg : Outport  Port=244
  VOUTP_SPTGDet_flg : Outport  Port=245
  VOUTP_APSOpenPTG_flg : Outport  Port=246
  VOUTP_FollowMe_flg : Outport  Port=247
  VOUTP_IVIRST_flg : Outport  Port=248
  VOUTP_CountAlarm_enum : Outport  Port=249
  VOUTP_MFSWTri_flg : Outport  Port=250
  VOUTP_MirrorFlodPos_flg : Outport  Port=251
  VOUTP_FuelDoorPos_flg : Outport  Port=252
  VOUTP_MFRDNBrightReq_pct : Outport  Port=253
  VOUTP_PTGInnerSW2_enum : Outport  Port=254
  VOUTP_DrvWdwCtrlCmd_pct : Outport  Port=255
  VOUTP_PasWdwCtrlCmd_pct : Outport  Port=256
  VOUTP_DrRWdwCtrlCmd_pct : Outport  Port=257
  VOUTP_PsRWdwCtrlCmd_pct : Outport  Port=258
  VOUTP_APMDoorControlSta_flg : Outport  Port=259
  VOUTP_AmbFunEN_flg : Outport  Port=260
  VOUTP_AmbWelEN_flg : Outport  Port=261
  VOUTP_AmbDimEN_flg : Outport  Port=262
  VOUTP_AmbLinkDriSta_flg : Outport  Port=263
  VOUTP_AmbPwrWarnEN_flg : Outport  Port=264
  VOUTP_AmbODAEN_flg : Outport  Port=265
  VOUTP_AmbColorSta_enum : Outport  Port=266
  VOUTP_AmbBrightSta_enum : Outport  Port=267
  VOUTP_LockAlarm_enum : Outport  Port=268
  VOUTP_ATCtrl_enum : Outport  Port=269
  VOUTP_fUnlockSingle_flg : Outport  Port=270
  VOUTP_UserNow_enum : Outport  Port=271
  VOUTP_AmbFunENFlash_enum : Outport  Port=272
  VOUTP_AmbWelENFlash_enum : Outport  Port=273
  VOUTP_AmbDimENFlash_enum : Outport  Port=274
  VOUTP_AmbLinkDriStaFlash_enum : Outport  Port=275
  VOUTP_AmbPwrWarnENFlash_enum : Outport  Port=276
  VOUTP_AmbODAENFlash_enum : Outport  Port=277
  VOUTP_AmbColorSta1_enum : Outport  Port=278
  VOUTP_AmbColorSta2_enum : Outport  Port=279
  VOUTP_AmbColorSta3_enum : Outport  Port=280
  VOUTP_AmbColorSta4_enum : Outport  Port=281
  VOUTP_AmbColorSta5_enum : Outport  Port=282
  VOUTP_AmbColorSta7_enum : Outport  Port=283
  VOUTP_AmbBrightnessSta1_enum : Outport  Port=284
  VOUTP_AmbBrightnessSta2_enum : Outport  Port=285
  VOUTP_AmbBrightnessSta3_enum : Outport  Port=286
  VOUTP_AmbBrightnessSta4_enum : Outport  Port=287
  VOUTP_AmbBrightnessSta5_enum : Outport  Port=288
  VOUTP_AmbBrightnessSta7_enum : Outport  Port=289
  VOUTP_HazardIND_flg : Outport  Port=290
  VOUTP_DimSwSta_flg : Outport  Port=291
  VOUTP_PassSWSta_flg : Outport  Port=292
  VOUTP_FWipSwSta_enum : Outport  Port=293
  VOUTP_FWasSwSta_enum : Outport  Port=294
  VOUTP_TurnSwSta_enum : Outport  Port=295
  VOUTP_TurnSwTSetSta_enum : Outport  Port=296
  VOUTP_SPTGENFun_flg : Outport  Port=297
  VOUTP_SPTGENFunMem_enum : Outport  Port=298
  VOUTP_OutMode_enum : Outport  Port=299
  VOUTP_TurnSwTimeSetSta123_enum : Outport  Port=300
  VOUTP_TurnSwTimeSetSta457_enum : Outport  Port=301
  VOUTP_FDLHandleLampCmd_flg : Outport  Port=302
  VOUTP_FDRHandleLampCmd_flg : Outport  Port=303
  VOUTP_FDHandleCmd_enum : Outport  Port=304
  VOUTP_HBeamADB_flg : Outport  Port=305
  VOUTP_WalkInUnLkENMem_enum : Outport  Port=306
  VOUTP_WalkOutLkENMem_enum : Outport  Port=307
  VOUTP_RmLpModeENMem_enum : Outport  Port=308
  VOUTP_LockSettingStaMem_enum : Outport  Port=309
  VOUTP_FollowMeENMem_enum : Outport  Port=310
  VOUTP_WalkInUnLkENFunSta_flg : Outport  Port=311
  VOUTP_WalkOutLkENFunSta_flg : Outport  Port=312
  VOUTP_RmLpModeENFunSta_flg : Outport  Port=313
  VOUTP_FollowMeENFunSta_flg : Outport  Port=314
  VOUTP_HoodRelCmd_flg : Outport  Port=315
  VOUTP_WelcomeLight_enum : Outport  Port=316
  VOUTP_PTGOpenHeightSta_enum : Outport  Port=317
  VOUTP_UserHeightSet_cnt : Outport  Port=318
  VOUTP_PTGUserHeight1_cnt : Outport  Port=319
  VOUTP_PTGUserHeight2_cnt : Outport  Port=320
  VOUTP_PTGUserHeight3_cnt : Outport  Port=321
  VOUTP_PTGUserHeight4_cnt : Outport  Port=322
  VOUTP_PTGUserHeight5_cnt : Outport  Port=323
  VOUTP_PTGUserHeight7_cnt : Outport  Port=324
  VOUTP_PTGOpenHeight12_enum : Outport  Port=325
  VOUTP_PTGOpenHeight34_enum : Outport  Port=326
  VOUTP_PTGOpenHeight57_enum : Outport  Port=327
  VOUTP_SenstivityPosnCmd_enum : Outport  Port=328
  VOUTP_TimeGapLevelSta_enum : Outport  Port=329
  VOUTP_ACCLevelMem12_enum : Outport  Port=330
  VOUTP_ACCLevelMem34_enum : Outport  Port=331
  VOUTP_ACCLevelMem57_enum : Outport  Port=332
  VOUTP_LRightStaCmd_flg : Outport  Port=333
  VOUTP_LLeftStaCmd_flg : Outport  Port=334
  VOUTP_AutoLockSta_flg : Outport  Port=335
  VOUTP_AutoLockMem_enum : Outport  Port=336
  VOUTP_AutoUnlockSta_flg : Outport  Port=337
  VOUTP_AutoUnlockMem_enum : Outport  Port=338
  VOUTP_HMIKey1FuncSta_enum : Outport  Port=339
  VOUTP_HMIKey2FuncSta_enum : Outport  Port=340
  VOUTP_HMIKey3FuncSta_enum : Outport  Port=341
  VOUTP_HMIKey4FuncSta_enum : Outport  Port=342
  VOUTP_HMIKey5FuncSta_enum : Outport  Port=343
  VOUTP_HMIKey6FuncSta_enum : Outport  Port=344
  VOUTP_HMIKey7FuncSta_enum : Outport  Port=345
  VOUTP_HMIKey8FuncSta_enum : Outport  Port=346
  VOUTP_AutoWipHSpdENSta_flg : Outport  Port=347
  VOUTP_DrvWdwReqAP_enum : Outport  Port=348
  VOUTP_PasWdwReqAP_enum : Outport  Port=349
  VOUTP_DrRWdwReqAP_enum : Outport  Port=350
  VOUTP_PsRWdwReqAP_enum : Outport  Port=351
  VOUTP_CLWinLockDrSta_flg : Outport  Port=352
  VOUTP_CLWinLockDrStaMem_enum : Outport  Port=353
  VOUTP_WinLFOpenedSta_pct : Outport  Port=354
  VOUTP_WinRFOpenedSta_pct : Outport  Port=355
  VOUTP_WinLROpenedSta_pct : Outport  Port=356
  VOUTP_WinRROpenedSta_pct : Outport  Port=357
  VOUTP_FoxPiSwitchSta_enum : Outport  Port=358
  VOUTP_FoxPiLampSta_enum : Outport  Port=359
  VOUTP_C3BMS6RCDTC_raw32 : Outport  Port=360
  VOUTP_C3BMS6CSDTC_raw32 : Outport  Port=361
  VOUTP_C3BMS6LCDTC_raw32 : Outport  Port=362
  VOUTP_C3BMS1RCDTC_raw32 : Outport  Port=363
  VOUTP_C3BMS1CSDTC_raw32 : Outport  Port=364
  VOUTP_C3BMS1LCDTC_raw32 : Outport  Port=365
  VOUTP_C3CCU1RCDTC_raw32 : Outport  Port=366
  VOUTP_C3CCU1CSDTC_raw32 : Outport  Port=367
  VOUTP_C3CCU1LCDTC_raw32 : Outport  Port=368
  VOUTP_C3CCU2RCDTC_raw32 : Outport  Port=369
  VOUTP_C3CCU2CSDTC_raw32 : Outport  Port=370
  VOUTP_C3CCU2LCDTC_raw32 : Outport  Port=371
  VOUTP_C1ABM1RCDTC_raw32 : Outport  Port=372
  VOUTP_C1ABM1CSDTC_raw32 : Outport  Port=373
  VOUTP_C1ABM1LCDTC_raw32 : Outport  Port=374
  VOUTP_Lv1ErrDTC_raw32 : Outport  Port=375
  VOUTP_Lv2ErrDTC_raw32 : Outport  Port=376
  VOUTP_Lv3ErrDTC_raw32 : Outport  Port=377
  VOUTP_Lv4ErrDTC_raw32 : Outport  Port=378
  VOUTP_BrkSWErrDTC_raw32 : Outport  Port=379
  VOUTP_BrkSWNoBacDTC_raw32 : Outport  Port=380
  VOUTP_KeyAuthDTC_raw32 : Outport  Port=381
  VOUTP_ONtoRdyDTC_raw32 : Outport  Port=382
  VOUTP_HVB4PreDTC_raw32 : Outport  Port=383
  VOUTP_MCU4PreDTC_raw32 : Outport  Port=384
  VOUTP_DCDC4PreDTC_raw32 : Outport  Port=385
  VOUTP_HVRlyCloDTC_raw32 : Outport  Port=386
  VOUTP_BMSRdyDTC_raw32 : Outport  Port=387
  VOUTP_DCDCEnaDTC_raw32 : Outport  Port=388
  VOUTP_HiLvSaChkDTC_raw32 : Outport  Port=389
  VOUTP_MidLvSaChkDTC_raw32 : Outport  Port=390
  VOUTP_MCUDisDTC_raw32 : Outport  Port=391
  VOUTP_DCDCDisDTC_raw32 : Outport  Port=392
  VOUTP_HVRlyOpDTC_raw32 : Outport  Port=393
  VOUTP_MCUActDTC_raw32 : Outport  Port=394
  VOUTP_OBC4PreDTC_raw32 : Outport  Port=395
  VOUTP_IniLVLoDTC_raw32 : Outport  Port=396
  VOUTP_LVSupLoDTC_raw32 : Outport  Port=397
  VOUTP_LVSupHiDTC_raw32 : Outport  Port=398
  VOUTP_DrStSWDTC_raw32 : Outport  Port=399
  VOUTP_FLDoorSWDTC_raw32 : Outport  Port=400
  VOUTP_RLDoorSWDTC_raw32 : Outport  Port=401
  VOUTP_FRDoorSWDTC_raw32 : Outport  Port=402
  VOUTP_RRDoorSWDTC_raw32 : Outport  Port=403
  VOUTP_HoodSWDTC_raw32 : Outport  Port=404
  VOUTP_TailgaSWDTC_raw32 : Outport  Port=405
  VOUTP_EDriveSysErrVCUErr_flg : Outport  Port=406
  VOUTP_VehMalfunLevel_enum : Outport  Port=407
  VOUTP_APS1SigOoRDTC_raw32 : Outport  Port=408
  VOUTP_APS2SigOoRDTC_raw32 : Outport  Port=409
  VOUTP_APSCorrErrDTC_raw32 : Outport  Port=410
  VOUTP_MCUF1NoComDTC_raw32 : Outport  Port=411
  VOUTP_MCUR1NoComDTC_raw32 : Outport  Port=412
  VOUTP_Shifter1NoComDTC_raw32 : Outport  Port=413
  VOUTP_ESC7NoComDTC_raw32 : Outport  Port=414
  VOUTP_ESC1NoComDTC_raw32 : Outport  Port=415
  VOUTP_ESC5NoComDTC_raw32 : Outport  Port=416
  VOUTP_EnterNewOperCyc_flg : Outport  Port=417
  VOUTP_DiagHCrashDTC_raw32 : Outport  Port=418
  VOUTP_DiagFLTSDTC_raw32 : Outport  Port=419
  VOUTP_DiagFRTSDTC_raw32 : Outport  Port=420
  VOUTP_DiagRLTSDTC_raw32 : Outport  Port=421
  VOUTP_DiagRRTSDTC_raw32 : Outport  Port=422
  VOUTP_FCLUSSDTC_raw32 : Outport  Port=423
  VOUTP_FMLUSSDTC_raw32 : Outport  Port=424
  VOUTP_FMRUSSDTC_raw32 : Outport  Port=425
  VOUTP_FCRUSSDTC_raw32 : Outport  Port=426
  VOUTP_RCLUSSDTC_raw32 : Outport  Port=427
  VOUTP_RMLUSSDTC_raw32 : Outport  Port=428
  VOUTP_RMRUSSDTC_raw32 : Outport  Port=429
  VOUTP_RCRUSSDTC_raw32 : Outport  Port=430
  VOUTP_FLLUSSDTC_raw32 : Outport  Port=431
  VOUTP_FLRUSSDTC_raw32 : Outport  Port=432
  VOUTP_RLLUSSDTC_raw32 : Outport  Port=433
  VOUTP_RLRUSSDTC_raw32 : Outport  Port=434
  VOUTP_FCM2NoComDTC_raw32 : Outport  Port=435
  VOUTP_FCM2RCErrDTC_raw32 : Outport  Port=436
  VOUTP_FCM2CSErrDTC_raw32 : Outport  Port=437
  VOUTP_FCM3NoComDTC_raw32 : Outport  Port=438
  VOUTP_FCM3RCErrDTC_raw32 : Outport  Port=439
  VOUTP_FCM3CSErrDTC_raw32 : Outport  Port=440
  VOUTP_FCM4NoComDTC_raw32 : Outport  Port=441
  VOUTP_FCM4CSErrDTC_raw32 : Outport  Port=442
  VOUTP_FCM5NoComDTC_raw32 : Outport  Port=443
  VOUTP_FCM5CSErrDTC_raw32 : Outport  Port=444
  VOUTP_ZoneSCPNoComDTC_raw32 : Outport  Port=445
  VOUTP_BMSSigErrDetDTC_raw32 : Outport  Port=446
  VOUTP_FCMACCSigErrDetDTC_raw32 : Outport  Port=447
  VOUTP_FrMCUSigErrDetDTC_raw32 : Outport  Port=448
  VOUTP_RrMCUSigErrDetDTC_raw32 : Outport  Port=449
  VOUTP_CCUSigErrDetDTC_raw32 : Outport  Port=450
  VOUTP_ACCAccelCmdErrDetDTC_raw32 : Outport  Port=451
  VOUTP_ACCMalfuncDetDTC_raw32 : Outport  Port=452
  VOUTP_CCMalfuncDetDTC_raw32 : Outport  Port=453
  VOUTP_MSAMalfuncDetDTC_raw32 : Outport  Port=454
  VOUTP_ISAMalfuncDetDTC_raw32 : Outport  Port=455
  VOUTP_MCUF1RCErrDTC_raw32 : Outport  Port=456
  VOUTP_MCUR1RCErrDTC_raw32 : Outport  Port=457
  VOUTP_MCUF1CSErrDTC_raw32 : Outport  Port=458
  VOUTP_MCUR1CSErrDTC_raw32 : Outport  Port=459
  VOUTP_Shifter1RCErrDTC_raw32 : Outport  Port=460
  VOUTP_Shifter1CSErrDTC_raw32 : Outport  Port=461
  VOUTP_ESC7RCErrDTC_raw32 : Outport  Port=462
  VOUTP_ESC7CSErrDTC_raw32 : Outport  Port=463
  VOUTP_ESC1RCErrDTC_raw32 : Outport  Port=464
  VOUTP_ESC1CSErrDTC_raw32 : Outport  Port=465
  VOUTP_ESC5RCErrDTC_raw32 : Outport  Port=466
  VOUTP_ESC5CSErrDTC_raw32 : Outport  Port=467
  VOUTP_FrMCUTqErrDTC_raw32 : Outport  Port=468
  VOUTP_RrMCUTqErrDTC_raw32 : Outport  Port=469
  VOUTP_LFBatwarnDTC_raw32 : Outport  Port=470
  VOUTP_RFBatwarnDTC_raw32 : Outport  Port=471
  VOUTP_LRBatwarnDTC_raw32 : Outport  Port=472
  VOUTP_RRBatwarnDTC_raw32 : Outport  Port=473
  VOUTP_LFPressIndiDTC_raw32 : Outport  Port=474
  VOUTP_RFPressIndiDTC_raw32 : Outport  Port=475
  VOUTP_LRPressIndiDTC_raw32 : Outport  Port=476
  VOUTP_RRPressIndiDTC_raw32 : Outport  Port=477
  VOUTP_LFWheelTmpHighDTC_raw32 : Outport  Port=478
  VOUTP_RFWheelTmpHighDTC_raw32 : Outport  Port=479
  VOUTP_LRWheelTmpHighDTC_raw32 : Outport  Port=480
  VOUTP_RRWheelTmpHighDTC_raw32 : Outport  Port=481
  VOUTP_LFSensorFailDTC_raw32 : Outport  Port=482
  VOUTP_RFSensorFailDTC_raw32 : Outport  Port=483
  VOUTP_LRSensorFailDTC_raw32 : Outport  Port=484
  VOUTP_RRSensorFailDTC_raw32 : Outport  Port=485
  VOUTP_C1EPAS2LCDTC_raw32 : Outport  Port=486
  VOUTP_5vAPS1PwrErrDTC_raw32 : Outport  Port=487
  VOUTP_5vAPS2PwrErrDTC_raw32 : Outport  Port=488
  VOUTP_EPBLockTODTC_raw32 : Outport  Port=489
  VOUTP_EPBUnlockTODTC_raw32 : Outport  Port=490
  VOUTP_LimpHomeActTmp_flg : Outport  Port=491
  VOUTP_DTCDetect_enum : Outport  Port=492
  VOUTP_EngagePFail_flg : Outport  Port=493
  VOUTP_DisengagePFail_flg : Outport  Port=494
  VOUTP_VCURAPSErrLv2_flg : Outport  Port=495
  VOUTP_VCURAPSErrLv3_flg : Outport  Port=496
